simulink model "nb_spectrometer_17"  (R2012b)
(part 2 of 148)

      mask prompts: PFBSize "Size of PFB: (2^? pnts)"; TotalTaps "Total Number of Taps:"; WindowType "Windowing Function:"; n_inputs "Number of Simultaneous Inputs: (2^?)"; MakeBiplex "Make Biplex?"; BitWidthIn "Input Bitwidth:"; BitWidthOut "Output Bitwidth:"; CoeffBitWidth "Coefficient Bitwidth:"; CoeffDistMem "Use Distributed Memory for Coeffs"; add_latency "Add Latency"; mult_latency "Mult Latency"; bram_latency "BRAM Latency"; fan_latency "Fanout latency"; conv_latency "Convert latency"; quantization "Quantization Behavior"; fwidth "Bin Width Scaling (normal=1)"; mult_spec "Multiplier specification (0=core, 1=embedded, 2=behavioural) (left=1st tap, or just one value)"; adder_folding "Fold adders into DSPs"; adder_imp "Adder implementation"; coeffs_share "Share coefficients between polarisations (use less BRAM)?"
      mask help:
      | Fold adders into DSPs: Causes adders to be absorbed into DSP blocks (supported in Virtex5)
      | Adder implementation: Cores using Fabric or DSP48 or behavioral HDL
      mask init:
      | pfb_fir_real_init(gcb, ...
      |     'PFBSize', PFBSize, ...
      |     'TotalTaps', TotalTaps, ...
      |     'WindowType', WindowType, ...
      |     'n_inputs', n_inputs, ...
      |     'MakeBiplex', MakeBiplex, ...
      |     'BitWidthIn', BitWidthIn, ...
      |     'BitWidthOut', BitWidthOut, ...
      |     'CoeffBitWidth', CoeffBitWidth, ...
      |     'CoeffDistMem', CoeffDistMem, ...
      |     'add_latency', add_latency, ...
      |     'mult_latency', mult_latency, ...
      |     'bram_latency', bram_latency, ...
      |     'fan_latency', fan_latency, ...
      |     'conv_latency', conv_latency, ...
      |     'quantization', quantization, ...
      |     'fwidth', fwidth, ...
      |     'mult_spec', mult_spec, ...
      |     'adder_folding', adder_folding, ...
      |     'adder_imp', adder_imp, ...
      |     'coeffs_share', coeffs_share);
      settings: AttributesFormatString=taps=2, add_latency=1
      mask Help: eval('xlWeb(''http://casper.berkeley.edu/wiki/Pfb_fir_real'')')
      mask Callback TotalTaps:
      | %num_taps = eval(get_param(gcb, 'TotalTaps'));
      | %old_vec = eval(get_param(gcb, 'mult_spec'));=-0l
      | 
      | %vec = 2.*ones(1,num_taps);
      | %old_size = length(old_vec);
      | 
      | %if(old_size <= num_taps),
      | %    new_size = old_size;
      | %else,
      | %    new_size = num_taps;
      | %end
      | 
      | %for n = 1:new_size, vec(n) = old_vec(n); end
      | %set_param(gcb, 'mult_spec', mat2str(vec));
      mask TypeOptions WindowType: bartlett | barthannwin | blackman | blackmanharris | bohamwin | chebwin | flattopwin | gausswin | hamming | hann | kaiser | nuttallwin | parzenwin | rectwin | tukeywin | triang | userwindow
      mask TypeOptions quantization: Truncate | Round  (unbiased: +/- Inf) | Round  (unbiased: Even Values)
      mask TypeOptions adder_imp: Behavioral | Fabric | DSP48
  pfb_fir_real1 : Subsystem  Tag=casper:pfb_fir_real  AncestorBlock=casper_library_pfbs/pfb_fir_real  mask(pfb_fir_real){PFBSize=9, TotalTaps=2, WindowType=hamming, n_inputs=2, MakeBiplex=off, BitWidthIn=8, BitWidthOut=18, CoeffBitWidth=18, CoeffDistMem=off, add_latency=1, mult_latency=2, bram_latency=2, fan_latency=1, conv_latency=1, quantization=Round  (unbiased: Even Values), fwidth=1, mult_spec=2, adder_folding=on, adder_imp=Fabric, coeffs_share=off}
      mask prompts: PFBSize "Size of PFB: (2^? pnts)"; TotalTaps "Total Number of Taps:"; WindowType "Windowing Function:"; n_inputs "Number of Simultaneous Inputs: (2^?)"; MakeBiplex "Make Biplex?"; BitWidthIn "Input Bitwidth:"; BitWidthOut "Output Bitwidth:"; CoeffBitWidth "Coefficient Bitwidth:"; CoeffDistMem "Use Distributed Memory for Coeffs"; add_latency "Add Latency"; mult_latency "Mult Latency"; bram_latency "BRAM Latency"; fan_latency "Fanout latency"; conv_latency "Convert latency"; quantization "Quantization Behavior"; fwidth "Bin Width Scaling (normal=1)"; mult_spec "Multiplier specification (0=core, 1=embedded, 2=behavioural) (left=1st tap, or just one value)"; adder_folding "Fold adders into DSPs"; adder_imp "Adder implementation"; coeffs_share "Share coefficients between polarisations (use less BRAM)?"
      mask help:
      | Fold adders into DSPs: Causes adders to be absorbed into DSP blocks (supported in Virtex5)
      | Adder implementation: Cores using Fabric or DSP48 or behavioral HDL
      mask init: same as nb_spectrometer_17/pfb_fir_real
      settings: AttributesFormatString=taps=2, add_latency=1
      mask Help: eval('xlWeb(''http://casper.berkeley.edu/wiki/Pfb_fir_real'')')
      mask Callback TotalTaps:
      | %num_taps = eval(get_param(gcb, 'TotalTaps'));
      | %old_vec = eval(get_param(gcb, 'mult_spec'));=-0l
      | 
      | %vec = 2.*ones(1,num_taps);
      | %old_size = length(old_vec);
      | 
      | %if(old_size <= num_taps),
      | %    new_size = old_size;
      | %else,
      | %    new_size = num_taps;
      | %end
      | 
      | %for n = 1:new_size, vec(n) = old_vec(n); end
      | %set_param(gcb, 'mult_spec', mat2str(vec));
      mask TypeOptions WindowType: bartlett | barthannwin | blackman | blackmanharris | bohamwin | chebwin | flattopwin | gausswin | hamming | hann | kaiser | nuttallwin | parzenwin | rectwin | tukeywin | triang | userwindow
      mask TypeOptions quantization: Truncate | Round  (unbiased: +/- Inf) | Round  (unbiased: Even Values)
      mask TypeOptions adder_imp: Behavioral | Fabric | DSP48
  posedge : Subsystem  AncestorBlock=casper_library_misc/edge_detect  mask(edge_detect){edge=Rising, polarity=Active High, x_in=[0 0.08 0.08 0.16 0.16 0.24 0.24 0.32 0.32 0.4], y_in=[-1 -1  1  1  1  1  1  1  1  1], x_out=[0.6 0.68 0.68 0.76 0.76 0.84 0.84 0.92 0.92 1], y_out=[-1 -1  1  1 -1 -1 -1 -1 -1 -1]}
      mask prompts: edge "Edge Type"; polarity "Output Polarity"; x_in "Input X Positions"; y_in "Input Y Positions"; x_out "Output X Positions"; y_out "Output Y Positions"
      mask help: Output is active for one-cycle after each edge of the specified type (i.e. rising, falling or both).
      mask init:
      | edge_detect_init(gcb,...
      |     'edge',edge,...
      |     'polarity',polarity,...
      |     'x_in',x_in,...
      |     'x_out',x_out,...
      |     'y_in',y_in,...
      |     'y_out',y_out);
      | 
      | x_in_num=str2num(getfield(getfield(get_param(gcb,'UserData'),'parameters'),'x_in'));
      | x_out_num=str2num(getfield(getfield(get_param(gcb,'UserData'),'parameters'),'x_out'));
      | y_in_num=str2num(getfield(getfield(get_param(gcb,'UserData'),'parameters'),'y_in'));
      | y_out_num=str2num(getfield(getfield(get_param(gcb,'UserData'),'parameters'),'y_out'));
      settings: AttributesFormatString=|
      | rising edges
      | active high
      mask Help: Output is active for one-cycle after each edge of the specified type (i.e. rising, falling, or both).  Latency is zero.
      mask TypeOptions edge: Rising | Falling | Both
      mask TypeOptions polarity: Active High | Active Low
      mask Display:
      | plot(x_in_num,0.5+y_in_num*0.2);
      | plot(x_out_num,0.5+y_out_num*0.2);
  posedge1 : Subsystem  AncestorBlock=casper_library_misc/edge_detect  mask(edge_detect){edge=Rising, polarity=Active High, x_in=[0 0.08 0.08 0.16 0.16 0.24 0.24 0.32 0.32 0.4], y_in=[-1 -1  1  1  1  1  1  1  1  1], x_out=[0.6 0.68 0.68 0.76 0.76 0.84 0.84 0.92 0.92 1], y_out=[-1 -1  1  1 -1 -1 -1 -1 -1 -1]}
      mask prompts: edge "Edge Type"; polarity "Output Polarity"; x_in "Input X Positions"; y_in "Input Y Positions"; x_out "Output X Positions"; y_out "Output Y Positions"
      mask help: Output is active for one-cycle after each edge of the specified type (i.e. rising, falling or both).
      mask init: same as nb_spectrometer_17/posedge
      settings: AttributesFormatString=|
      | rising edges
      | active high
      mask Help: Output is active for one-cycle after each edge of the specified type (i.e. rising, falling, or both).  Latency is zero.
      mask TypeOptions edge: Rising | Falling | Both
      mask TypeOptions polarity: Active High | Active Low
      mask Display:
      | plot(x_in_num,0.5+y_in_num*0.2);
      | plot(x_out_num,0.5+y_out_num*0.2);
  posedge10 : Subsystem  AncestorBlock=casper_library_misc/edge_detect  mask(edge_detect){edge=Rising, polarity=Active High, x_in=[0 0.08 0.08 0.16 0.16 0.24 0.24 0.32 0.32 0.4], y_in=[-1 -1  1  1  1  1  1  1  1  1], x_out=[0.6 0.68 0.68 0.76 0.76 0.84 0.84 0.92 0.92 1], y_out=[-1 -1  1  1 -1 -1 -1 -1 -1 -1]}
      mask prompts: edge "Edge Type"; polarity "Output Polarity"; x_in "Input X Positions"; y_in "Input Y Positions"; x_out "Output X Positions"; y_out "Output Y Positions"
      mask help: Output is active for one-cycle after each edge of the specified type (i.e. rising, falling or both).
      mask init: same as nb_spectrometer_17/posedge
      settings: AttributesFormatString=|
      | rising edges
      | active high
      mask Help: Output is active for one-cycle after each edge of the specified type (i.e. rising, falling, or both).  Latency is zero.
      mask TypeOptions edge: Rising | Falling | Both
      mask TypeOptions polarity: Active High | Active Low
      mask Display:
      | plot(x_in_num,0.5+y_in_num*0.2);
      | plot(x_out_num,0.5+y_out_num*0.2);
  posedge11 : Subsystem  AncestorBlock=casper_library_misc/edge_detect  mask(edge_detect){edge=Rising, polarity=Active High, x_in=[0 0.08 0.08 0.16 0.16 0.24 0.24 0.32 0.32 0.4], y_in=[-1 -1  1  1  1  1  1  1  1  1], x_out=[0.6 0.68 0.68 0.76 0.76 0.84 0.84 0.92 0.92 1], y_out=[-1 -1  1  1 -1 -1 -1 -1 -1 -1]}
      mask prompts: edge "Edge Type"; polarity "Output Polarity"; x_in "Input X Positions"; y_in "Input Y Positions"; x_out "Output X Positions"; y_out "Output Y Positions"
      mask help: Output is active for one-cycle after each edge of the specified type (i.e. rising, falling or both).
      mask init: same as nb_spectrometer_17/posedge
      settings: AttributesFormatString=|
      | rising edges
      | active high
      mask Help: Output is active for one-cycle after each edge of the specified type (i.e. rising, falling, or both).  Latency is zero.
      mask TypeOptions edge: Rising | Falling | Both
      mask TypeOptions polarity: Active High | Active Low
      mask Display:
      | plot(x_in_num,0.5+y_in_num*0.2);
      | plot(x_out_num,0.5+y_out_num*0.2);
  posedge12 : Subsystem  AncestorBlock=casper_library_misc/edge_detect  mask(edge_detect){edge=Rising, polarity=Active High, x_in=[0 0.08 0.08 0.16 0.16 0.24 0.24 0.32 0.32 0.4], y_in=[-1 -1  1  1  1  1  1  1  1  1], x_out=[0.6 0.68 0.68 0.76 0.76 0.84 0.84 0.92 0.92 1], y_out=[-1 -1  1  1 -1 -1 -1 -1 -1 -1]}
      mask prompts: edge "Edge Type"; polarity "Output Polarity"; x_in "Input X Positions"; y_in "Input Y Positions"; x_out "Output X Positions"; y_out "Output Y Positions"
      mask help: Output is active for one-cycle after each edge of the specified type (i.e. rising, falling or both).
      mask init: same as nb_spectrometer_17/posedge
      settings: AttributesFormatString=|
      | rising edges
      | active high
      mask Help: Output is active for one-cycle after each edge of the specified type (i.e. rising, falling, or both).  Latency is zero.
      mask TypeOptions edge: Rising | Falling | Both
      mask TypeOptions polarity: Active High | Active Low
      mask Display:
      | plot(x_in_num,0.5+y_in_num*0.2);
      | plot(x_out_num,0.5+y_out_num*0.2);
  posedge13 : Subsystem  AncestorBlock=casper_library_misc/edge_detect  mask(edge_detect){edge=Rising, polarity=Active High, x_in=[0 0.08 0.08 0.16 0.16 0.24 0.24 0.32 0.32 0.4], y_in=[-1 -1  1  1  1  1  1  1  1  1], x_out=[0.6 0.68 0.68 0.76 0.76 0.84 0.84 0.92 0.92 1], y_out=[-1 -1  1  1 -1 -1 -1 -1 -1 -1]}
      mask prompts: edge "Edge Type"; polarity "Output Polarity"; x_in "Input X Positions"; y_in "Input Y Positions"; x_out "Output X Positions"; y_out "Output Y Positions"
      mask help: Output is active for one-cycle after each edge of the specified type (i.e. rising, falling or both).
      mask init: same as nb_spectrometer_17/posedge
      settings: AttributesFormatString=|
      | rising edges
      | active high
      mask Help: Output is active for one-cycle after each edge of the specified type (i.e. rising, falling, or both).  Latency is zero.
      mask TypeOptions edge: Rising | Falling | Both
      mask TypeOptions polarity: Active High | Active Low
      mask Display:
      | plot(x_in_num,0.5+y_in_num*0.2);
      | plot(x_out_num,0.5+y_out_num*0.2);
  posedge14 : Subsystem  AncestorBlock=casper_library_misc/edge_detect  mask(edge_detect){edge=Rising, polarity=Active High, x_in=[0 0.08 0.08 0.16 0.16 0.24 0.24 0.32 0.32 0.4], y_in=[-1 -1  1  1  1  1  1  1  1  1], x_out=[0.6 0.68 0.68 0.76 0.76 0.84 0.84 0.92 0.92 1], y_out=[-1 -1  1  1 -1 -1 -1 -1 -1 -1]}
      mask prompts: edge "Edge Type"; polarity "Output Polarity"; x_in "Input X Positions"; y_in "Input Y Positions"; x_out "Output X Positions"; y_out "Output Y Positions"
      mask help: Output is active for one-cycle after each edge of the specified type (i.e. rising, falling or both).
      mask init: same as nb_spectrometer_17/posedge
      settings: AttributesFormatString=|
      | rising edges
      | active high
      mask Help: Output is active for one-cycle after each edge of the specified type (i.e. rising, falling, or both).  Latency is zero.
      mask TypeOptions edge: Rising | Falling | Both
      mask TypeOptions polarity: Active High | Active Low
      mask Display:
      | plot(x_in_num,0.5+y_in_num*0.2);
      | plot(x_out_num,0.5+y_out_num*0.2);
  posedge15 : Subsystem  AncestorBlock=casper_library_misc/edge_detect  mask(edge_detect){edge=Rising, polarity=Active High, x_in=[0 0.08 0.08 0.16 0.16 0.24 0.24 0.32 0.32 0.4], y_in=[-1 -1  1  1  1  1  1  1  1  1], x_out=[0.6 0.68 0.68 0.76 0.76 0.84 0.84 0.92 0.92 1], y_out=[-1 -1  1  1 -1 -1 -1 -1 -1 -1]}
      mask prompts: edge "Edge Type"; polarity "Output Polarity"; x_in "Input X Positions"; y_in "Input Y Positions"; x_out "Output X Positions"; y_out "Output Y Positions"
      mask help: Output is active for one-cycle after each edge of the specified type (i.e. rising, falling or both).
      mask init: same as nb_spectrometer_17/posedge
      settings: AttributesFormatString=|
      | rising edges
      | active high
      mask Help: Output is active for one-cycle after each edge of the specified type (i.e. rising, falling, or both).  Latency is zero.
      mask TypeOptions edge: Rising | Falling | Both
      mask TypeOptions polarity: Active High | Active Low
      mask Display:
      | plot(x_in_num,0.5+y_in_num*0.2);
      | plot(x_out_num,0.5+y_out_num*0.2);
  posedge16 : Subsystem  AncestorBlock=casper_library_misc/edge_detect  mask(edge_detect){edge=Rising, polarity=Active High, x_in=[0 0.08 0.08 0.16 0.16 0.24 0.24 0.32 0.32 0.4], y_in=[-1 -1  1  1  1  1  1  1  1  1], x_out=[0.6 0.68 0.68 0.76 0.76 0.84 0.84 0.92 0.92 1], y_out=[-1 -1  1  1 -1 -1 -1 -1 -1 -1]}
      mask prompts: edge "Edge Type"; polarity "Output Polarity"; x_in "Input X Positions"; y_in "Input Y Positions"; x_out "Output X Positions"; y_out "Output Y Positions"
      mask help: Output is active for one-cycle after each edge of the specified type (i.e. rising, falling or both).
      mask init: same as nb_spectrometer_17/posedge
      settings: AttributesFormatString=|
      | rising edges
      | active high
      mask Help: Output is active for one-cycle after each edge of the specified type (i.e. rising, falling, or both).  Latency is zero.
      mask TypeOptions edge: Rising | Falling | Both
      mask TypeOptions polarity: Active High | Active Low
      mask Display:
      | plot(x_in_num,0.5+y_in_num*0.2);
      | plot(x_out_num,0.5+y_out_num*0.2);
  posedge17 : Subsystem  AncestorBlock=casper_library_misc/edge_detect  mask(edge_detect){edge=Falling, polarity=Active High, x_in=[0 0.08 0.08 0.16 0.16 0.24 0.24 0.32 0.32 0.4], y_in=[-1 -1  1  1  1  1  1  1  1  1], x_out=[0.6 0.68 0.68 0.76 0.76 0.84 0.84 0.92 0.92 1], y_out=[-1 -1  1  1 -1 -1 -1 -1 -1 -1]}
      mask prompts: edge "Edge Type"; polarity "Output Polarity"; x_in "Input X Positions"; y_in "Input Y Positions"; x_out "Output X Positions"; y_out "Output Y Positions"
      mask help: Output is active for one-cycle after each edge of the specified type (i.e. rising, falling or both).
      mask init: same as nb_spectrometer_17/posedge
      settings: AttributesFormatString=|
      | falling edges
      | active high
      mask Help: Output is active for one-cycle after each edge of the specified type (i.e. rising, falling, or both).  Latency is zero.
      mask TypeOptions edge: Rising | Falling | Both
      mask TypeOptions polarity: Active High | Active Low
      mask Display:
      | plot(x_in_num,0.5+y_in_num*0.2);
      | plot(x_out_num,0.5+y_out_num*0.2);
  posedge18 : Subsystem  AncestorBlock=casper_library_misc/edge_detect  mask(edge_detect){edge=Rising, polarity=Active High, x_in=[0 0.08 0.08 0.16 0.16 0.24 0.24 0.32 0.32 0.4], y_in=[-1 -1  1  1  1  1  1  1  1  1], x_out=[0.6 0.68 0.68 0.76 0.76 0.84 0.84 0.92 0.92 1], y_out=[-1 -1  1  1 -1 -1 -1 -1 -1 -1]}
      mask prompts: edge "Edge Type"; polarity "Output Polarity"; x_in "Input X Positions"; y_in "Input Y Positions"; x_out "Output X Positions"; y_out "Output Y Positions"
      mask help: Output is active for one-cycle after each edge of the specified type (i.e. rising, falling or both).
      mask init: same as nb_spectrometer_17/posedge
      settings: AttributesFormatString=|
      | rising edges
      | active high
      mask Help: Output is active for one-cycle after each edge of the specified type (i.e. rising, falling, or both).  Latency is zero.
      mask TypeOptions edge: Rising | Falling | Both
      mask TypeOptions polarity: Active High | Active Low
      mask Display:
      | plot(x_in_num,0.5+y_in_num*0.2);
      | plot(x_out_num,0.5+y_out_num*0.2);
  posedge19 : Subsystem  AncestorBlock=casper_library_misc/edge_detect  mask(edge_detect){edge=Rising, polarity=Active High, x_in=[0 0.08 0.08 0.16 0.16 0.24 0.24 0.32 0.32 0.4], y_in=[-1 -1  1  1  1  1  1  1  1  1], x_out=[0.6 0.68 0.68 0.76 0.76 0.84 0.84 0.92 0.92 1], y_out=[-1 -1  1  1 -1 -1 -1 -1 -1 -1]}
      mask prompts: edge "Edge Type"; polarity "Output Polarity"; x_in "Input X Positions"; y_in "Input Y Positions"; x_out "Output X Positions"; y_out "Output Y Positions"
      mask help: Output is active for one-cycle after each edge of the specified type (i.e. rising, falling or both).
      mask init: same as nb_spectrometer_17/posedge
      settings: AttributesFormatString=|
      | rising edges
      | active high
      mask Help: Output is active for one-cycle after each edge of the specified type (i.e. rising, falling, or both).  Latency is zero.
      mask TypeOptions edge: Rising | Falling | Both
      mask TypeOptions polarity: Active High | Active Low
      mask Display:
      | plot(x_in_num,0.5+y_in_num*0.2);
      | plot(x_out_num,0.5+y_out_num*0.2);
  posedge2 : Subsystem  AncestorBlock=casper_library_misc/edge_detect  mask(edge_detect){edge=Rising, polarity=Active High, x_in=[0 0.08 0.08 0.16 0.16 0.24 0.24 0.32 0.32 0.4], y_in=[-1 -1  1  1  1  1  1  1  1  1], x_out=[0.6 0.68 0.68 0.76 0.76 0.84 0.84 0.92 0.92 1], y_out=[-1 -1  1  1 -1 -1 -1 -1 -1 -1]}
      mask prompts: edge "Edge Type"; polarity "Output Polarity"; x_in "Input X Positions"; y_in "Input Y Positions"; x_out "Output X Positions"; y_out "Output Y Positions"
      mask help: Output is active for one-cycle after each edge of the specified type (i.e. rising, falling or both).
      mask init: same as nb_spectrometer_17/posedge
      settings: AttributesFormatString=|
      | rising edges
      | active high
      mask Help: Output is active for one-cycle after each edge of the specified type (i.e. rising, falling, or both).  Latency is zero.
      mask TypeOptions edge: Rising | Falling | Both
      mask TypeOptions polarity: Active High | Active Low
      mask Display:
      | plot(x_in_num,0.5+y_in_num*0.2);
      | plot(x_out_num,0.5+y_out_num*0.2);
  posedge20 : Subsystem  AncestorBlock=casper_library_misc/edge_detect  mask(edge_detect){edge=Rising, polarity=Active High, x_in=[0 0.08 0.08 0.16 0.16 0.24 0.24 0.32 0.32 0.4], y_in=[-1 -1  1  1  1  1  1  1  1  1], x_out=[0.6 0.68 0.68 0.76 0.76 0.84 0.84 0.92 0.92 1], y_out=[-1 -1  1  1 -1 -1 -1 -1 -1 -1]}
      mask prompts: edge "Edge Type"; polarity "Output Polarity"; x_in "Input X Positions"; y_in "Input Y Positions"; x_out "Output X Positions"; y_out "Output Y Positions"
      mask help: Output is active for one-cycle after each edge of the specified type (i.e. rising, falling or both).
      mask init: same as nb_spectrometer_17/posedge
      settings: AttributesFormatString=|
      | rising edges
      | active high
      mask Help: Output is active for one-cycle after each edge of the specified type (i.e. rising, falling, or both).  Latency is zero.
      mask TypeOptions edge: Rising | Falling | Both
      mask TypeOptions polarity: Active High | Active Low
      mask Display:
      | plot(x_in_num,0.5+y_in_num*0.2);
      | plot(x_out_num,0.5+y_out_num*0.2);
  posedge3 : Subsystem  AncestorBlock=casper_library_misc/edge_detect  mask(edge_detect){edge=Rising, polarity=Active High, x_in=[0 0.08 0.08 0.16 0.16 0.24 0.24 0.32 0.32 0.4], y_in=[-1 -1  1  1  1  1  1  1  1  1], x_out=[0.6 0.68 0.68 0.76 0.76 0.84 0.84 0.92 0.92 1], y_out=[-1 -1  1  1 -1 -1 -1 -1 -1 -1]}
      mask prompts: edge "Edge Type"; polarity "Output Polarity"; x_in "Input X Positions"; y_in "Input Y Positions"; x_out "Output X Positions"; y_out "Output Y Positions"
      mask help: Output is active for one-cycle after each edge of the specified type (i.e. rising, falling or both).
      mask init: same as nb_spectrometer_17/posedge
      settings: AttributesFormatString=|
      | rising edges
      | active high
      mask Help: Output is active for one-cycle after each edge of the specified type (i.e. rising, falling, or both).  Latency is zero.
      mask TypeOptions edge: Rising | Falling | Both
      mask TypeOptions polarity: Active High | Active Low
      mask Display:
      | plot(x_in_num,0.5+y_in_num*0.2);
      | plot(x_out_num,0.5+y_out_num*0.2);
  posedge4 : Subsystem  AncestorBlock=casper_library_misc/edge_detect  mask(edge_detect){edge=Rising, polarity=Active High, x_in=[0 0.08 0.08 0.16 0.16 0.24 0.24 0.32 0.32 0.4], y_in=[-1 -1  1  1  1  1  1  1  1  1], x_out=[0.6 0.68 0.68 0.76 0.76 0.84 0.84 0.92 0.92 1], y_out=[-1 -1  1  1 -1 -1 -1 -1 -1 -1]}
      mask prompts: edge "Edge Type"; polarity "Output Polarity"; x_in "Input X Positions"; y_in "Input Y Positions"; x_out "Output X Positions"; y_out "Output Y Positions"
      mask help: Output is active for one-cycle after each edge of the specified type (i.e. rising, falling or both).
      mask init: same as nb_spectrometer_17/posedge
      settings: AttributesFormatString=|
      | rising edges
      | active high
      mask Help: Output is active for one-cycle after each edge of the specified type (i.e. rising, falling, or both).  Latency is zero.
      mask TypeOptions edge: Rising | Falling | Both
      mask TypeOptions polarity: Active High | Active Low
      mask Display:
      | plot(x_in_num,0.5+y_in_num*0.2);
      | plot(x_out_num,0.5+y_out_num*0.2);
  posedge5 : Subsystem  AncestorBlock=casper_library_misc/edge_detect  mask(edge_detect){edge=Rising, polarity=Active High, x_in=[0 0.08 0.08 0.16 0.16 0.24 0.24 0.32 0.32 0.4], y_in=[-1 -1  1  1  1  1  1  1  1  1], x_out=[0.6 0.68 0.68 0.76 0.76 0.84 0.84 0.92 0.92 1], y_out=[-1 -1  1  1 -1 -1 -1 -1 -1 -1]}
      mask prompts: edge "Edge Type"; polarity "Output Polarity"; x_in "Input X Positions"; y_in "Input Y Positions"; x_out "Output X Positions"; y_out "Output Y Positions"
      mask help: Output is active for one-cycle after each edge of the specified type (i.e. rising, falling or both).
      mask init: same as nb_spectrometer_17/posedge
      settings: AttributesFormatString=|
      | rising edges
      | active high
      mask Help: Output is active for one-cycle after each edge of the specified type (i.e. rising, falling, or both).  Latency is zero.
      mask TypeOptions edge: Rising | Falling | Both
      mask TypeOptions polarity: Active High | Active Low
      mask Display:
      | plot(x_in_num,0.5+y_in_num*0.2);
      | plot(x_out_num,0.5+y_out_num*0.2);
  posedge6 : Subsystem  AncestorBlock=casper_library_misc/edge_detect  mask(edge_detect){edge=Rising, polarity=Active High, x_in=[0 0.08 0.08 0.16 0.16 0.24 0.24 0.32 0.32 0.4], y_in=[-1 -1  1  1  1  1  1  1  1  1], x_out=[0.6 0.68 0.68 0.76 0.76 0.84 0.84 0.92 0.92 1], y_out=[-1 -1  1  1 -1 -1 -1 -1 -1 -1]}
      mask prompts: edge "Edge Type"; polarity "Output Polarity"; x_in "Input X Positions"; y_in "Input Y Positions"; x_out "Output X Positions"; y_out "Output Y Positions"
      mask help: Output is active for one-cycle after each edge of the specified type (i.e. rising, falling or both).
      mask init: same as nb_spectrometer_17/posedge
      settings: AttributesFormatString=|
      | rising edges
      | active high
      mask Help: Output is active for one-cycle after each edge of the specified type (i.e. rising, falling, or both).  Latency is zero.
      mask TypeOptions edge: Rising | Falling | Both
      mask TypeOptions polarity: Active High | Active Low
      mask Display:
      | plot(x_in_num,0.5+y_in_num*0.2);
      | plot(x_out_num,0.5+y_out_num*0.2);
  posedge7 : Subsystem  AncestorBlock=casper_library_misc/edge_detect  mask(edge_detect){edge=Rising, polarity=Active High, x_in=[0 0.08 0.08 0.16 0.16 0.24 0.24 0.32 0.32 0.4], y_in=[-1 -1  1  1  1  1  1  1  1  1], x_out=[0.6 0.68 0.68 0.76 0.76 0.84 0.84 0.92 0.92 1], y_out=[-1 -1  1  1 -1 -1 -1 -1 -1 -1]}
      mask prompts: edge "Edge Type"; polarity "Output Polarity"; x_in "Input X Positions"; y_in "Input Y Positions"; x_out "Output X Positions"; y_out "Output Y Positions"
      mask help: Output is active for one-cycle after each edge of the specified type (i.e. rising, falling or both).
      mask init: same as nb_spectrometer_17/posedge
      settings: AttributesFormatString=|
      | rising edges
      | active high
      mask Help: Output is active for one-cycle after each edge of the specified type (i.e. rising, falling, or both).  Latency is zero.
      mask TypeOptions edge: Rising | Falling | Both
      mask TypeOptions polarity: Active High | Active Low
      mask Display:
      | plot(x_in_num,0.5+y_in_num*0.2);
      | plot(x_out_num,0.5+y_out_num*0.2);
  posedge8 : Subsystem  AncestorBlock=casper_library_misc/edge_detect  mask(edge_detect){edge=Rising, polarity=Active High, x_in=[0 0.08 0.08 0.16 0.16 0.24 0.24 0.32 0.32 0.4], y_in=[-1 -1  1  1  1  1  1  1  1  1], x_out=[0.6 0.68 0.68 0.76 0.76 0.84 0.84 0.92 0.92 1], y_out=[-1 -1  1  1 -1 -1 -1 -1 -1 -1]}
      mask prompts: edge "Edge Type"; polarity "Output Polarity"; x_in "Input X Positions"; y_in "Input Y Positions"; x_out "Output X Positions"; y_out "Output Y Positions"
      mask help: Output is active for one-cycle after each edge of the specified type (i.e. rising, falling or both).
      mask init: same as nb_spectrometer_17/posedge
      settings: AttributesFormatString=|
      | rising edges
      | active high
      mask Help: Output is active for one-cycle after each edge of the specified type (i.e. rising, falling, or both).  Latency is zero.
      mask TypeOptions edge: Rising | Falling | Both
      mask TypeOptions polarity: Active High | Active Low
      mask Display:
      | plot(x_in_num,0.5+y_in_num*0.2);
      | plot(x_out_num,0.5+y_out_num*0.2);
  posedge9 : Subsystem  AncestorBlock=casper_library_misc/edge_detect  mask(edge_detect){edge=Rising, polarity=Active High, x_in=[0 0.08 0.08 0.16 0.16 0.24 0.24 0.32 0.32 0.4], y_in=[-1 -1  1  1  1  1  1  1  1  1], x_out=[0.6 0.68 0.68 0.76 0.76 0.84 0.84 0.92 0.92 1], y_out=[-1 -1  1  1 -1 -1 -1 -1 -1 -1]}
      mask prompts: edge "Edge Type"; polarity "Output Polarity"; x_in "Input X Positions"; y_in "Input Y Positions"; x_out "Output X Positions"; y_out "Output Y Positions"
      mask help: Output is active for one-cycle after each edge of the specified type (i.e. rising, falling or both).
      mask init: same as nb_spectrometer_17/posedge
      settings: AttributesFormatString=|
      | rising edges
      | active high
      mask Help: Output is active for one-cycle after each edge of the specified type (i.e. rising, falling, or both).  Latency is zero.
      mask TypeOptions edge: Rising | Falling | Both
      mask TypeOptions polarity: Active High | Active Low
      mask Display:
      | plot(x_in_num,0.5+y_in_num*0.2);
      | plot(x_out_num,0.5+y_out_num*0.2);
  pps_cnt : Subsystem  Tag=xps:sw_reg  AncestorBlock=xps_library/software register  mask(swreg){mode=one value, io_dir=To Processor, io_delay=0, sample_period=1, names=reg, bitwidths=32, arith_types=0, bin_pts=0, sim_port=on, show_format=off}
      mask prompts: io_dir "I/O direction"; io_delay "I/O delay"; sample_period "Sample period"; names "Name:"; bitwidths "Bitwidth:"; arith_types "Type (ufix=0, fix=1, bool=2):"; bin_pts "Binary pt:"; sim_port "Provide sim input/output?"; show_format "Print format string?"
      mask init:
      | swreg_init(gcb)
      settings: AttributesFormatString=1output
      mask TypeOptions mode: one value | fields of equal size | fields of arbitrary size
      mask Callback mode: swreg_cb(gcb);
      mask TypeOptions io_dir: To Processor | From Processor
      mask Callback io_dir:
      | mask_enables = get_param(gcb, 'MaskEnables');
      | mask_names = get_param(gcb, 'MaskNames');
      | if strcmp(get_param(gcb, 'io_dir'), 'To Processor'),
      |     mask_enables{ismember(mask_names, 'sample_period')} = 'off';
      | else
      |     mask_enables{ismember(mask_names, 'sample_period')} = 'on';
      | end
      | set_param(gcb, 'MaskEnables', mask_enables);
      mask Callback bitwidths: swreg_maskcheck(gcb);
      mask Callback arith_types: [numios, ~, ~, ~, current_types] = swreg_maskcheck(gcb);
      mask Callback bin_pts: swreg_maskcheck(gcb);
  pps_cnt1 : Subsystem  Tag=xps:sw_reg  Commented=on  AncestorBlock=xps_library/software register  mask(swreg){mode=one value, io_dir=To Processor, io_delay=0, sample_period=1, names=reg, bitwidths=32, arith_types=0, bin_pts=0, sim_port=on, show_format=off}
      mask prompts: io_dir "I/O direction"; io_delay "I/O delay"; sample_period "Sample period"; names "Name:"; bitwidths "Bitwidth:"; arith_types "Type (ufix=0, fix=1, bool=2):"; bin_pts "Binary pt:"; sim_port "Provide sim input/output?"; show_format "Print format string?"
      mask init:
      | swreg_init(gcb)
      settings: AttributesFormatString=1output
      mask TypeOptions mode: one value | fields of equal size | fields of arbitrary size
      mask Callback mode: swreg_cb(gcb);
      mask TypeOptions io_dir: To Processor | From Processor
      mask Callback io_dir:
      | mask_enables = get_param(gcb, 'MaskEnables');
      | mask_names = get_param(gcb, 'MaskNames');
      | if strcmp(get_param(gcb, 'io_dir'), 'To Processor'),
      |     mask_enables{ismember(mask_names, 'sample_period')} = 'off';
      | else
      |     mask_enables{ismember(mask_names, 'sample_period')} = 'on';
      | end
      | set_param(gcb, 'MaskEnables', mask_enables);
      mask Callback bitwidths: swreg_maskcheck(gcb);
      mask Callback arith_types: [numios, ~, ~, ~, current_types] = swreg_maskcheck(gcb);
      mask Callback bin_pts: swreg_maskcheck(gcb);
  pulse_ext{,1..6} (7 alike) : casper_library_misc/pulse_ext  pulse_len=20000000
  queue_empty : Subsystem  Tag=xps:sw_reg  AncestorBlock=xps_library/software register  mask(swreg){mode=one value, io_dir=To Processor, io_delay=0, sample_period=1, names=reg, bitwidths=1, arith_types=2, bin_pts=0, sim_port=on, show_format=off}
      mask prompts: io_dir "I/O direction"; io_delay "I/O delay"; sample_period "Sample period"; names "Name:"; bitwidths "Bitwidth:"; arith_types "Type (ufix=0, fix=1, bool=2):"; bin_pts "Binary pt:"; sim_port "Provide sim input/output?"; show_format "Print format string?"
      mask init:
      | swreg_init(gcb)
      settings: AttributesFormatString=1output
      mask TypeOptions mode: one value | fields of equal size | fields of arbitrary size
      mask Callback mode: swreg_cb(gcb);
      mask TypeOptions io_dir: To Processor | From Processor
      mask Callback io_dir:
      | mask_enables = get_param(gcb, 'MaskEnables');
      | mask_names = get_param(gcb, 'MaskNames');
      | if strcmp(get_param(gcb, 'io_dir'), 'To Processor'),
      |     mask_enables{ismember(mask_names, 'sample_period')} = 'off';
      | else
      |     mask_enables{ismember(mask_names, 'sample_period')} = 'on';
      | end
      | set_param(gcb, 'MaskEnables', mask_enables);
      mask Callback bitwidths: swreg_maskcheck(gcb);
      mask Callback arith_types: [numios, ~, ~, ~, current_types] = swreg_maskcheck(gcb);
      mask Callback bin_pts: swreg_maskcheck(gcb);
  queue_perc_full : Subsystem  Tag=xps:sw_reg  AncestorBlock=xps_library/software register  mask(swreg){mode=one value, io_dir=To Processor, io_delay=0, sample_period=1, names=reg, bitwidths=8, arith_types=0, bin_pts=8, sim_port=on, show_format=off}
      mask prompts: io_dir "I/O direction"; io_delay "I/O delay"; sample_period "Sample period"; names "Name:"; bitwidths "Bitwidth:"; arith_types "Type (ufix=0, fix=1, bool=2):"; bin_pts "Binary pt:"; sim_port "Provide sim input/output?"; show_format "Print format string?"
      mask init:
      | swreg_init(gcb)
      settings: AttributesFormatString=1output
      mask TypeOptions mode: one value | fields of equal size | fields of arbitrary size
      mask Callback mode: swreg_cb(gcb);
      mask TypeOptions io_dir: To Processor | From Processor
      mask Callback io_dir:
      | mask_enables = get_param(gcb, 'MaskEnables');
      | mask_names = get_param(gcb, 'MaskNames');
      | if strcmp(get_param(gcb, 'io_dir'), 'To Processor'),
      |     mask_enables{ismember(mask_names, 'sample_period')} = 'off';
      | else
      |     mask_enables{ismember(mask_names, 'sample_period')} = 'on';
      | end
      | set_param(gcb, 'MaskEnables', mask_enables);
      mask Callback bitwidths: swreg_maskcheck(gcb);
      mask Callback arith_types: [numios, ~, ~, ~, current_types] = swreg_maskcheck(gcb);
      mask Callback bin_pts: swreg_maskcheck(gcb);
  reinterpret10 : xbsIndex_r4/Reinterpret  force_arith_type=on  arith_type="Signed  (2's comp)"  force_bin_pt=on  bin_pt=0  block_type=reinterpret
  reinterpret11 : xbsIndex_r4/Reinterpret  force_arith_type=on  arith_type="Signed  (2's comp)"  force_bin_pt=on  bin_pt=0  block_type=reinterpret
  relational12 : xbsIndex_r4/Relational  mode=a>b  en=off  latency=1  dbl_ovrd=off  block_type=relational
  relational13 : xbsIndex_r4/Relational  mode=a<b  en=off  latency=1  dbl_ovrd=off  block_type=relational
  relational14 : xbsIndex_r4/Relational  mode=a>b  en=off  latency=0  dbl_ovrd=off  block_type=relational
  relational15 : xbsIndex_r4/Relational  mode=a>b  en=off  latency=1  dbl_ovrd=off  block_type=relational
  relational16 : xbsIndex_r4/Relational  mode=a<b  en=off  latency=1  dbl_ovrd=off  block_type=relational
  roach_gpio_a_enable_not : xps_library/gpio  Tag=xps:gpio  io_group=ROACH:gpioa_oe_n  io_dir=out  arith_type=Boolean  bitwidth=1  bin_pt=0  bit_index=0  sample_period=1  use_single_ended=off  use_ddr=off  reg_iob=off  reg_clk_phase=0  termination=None
      link override convert: arith_type=Boolean  n_bits=1  bin_pt=0
  roach_gpio_b_enable_not : xps_library/gpio  Tag=xps:gpio  io_group=ROACH:gpiob_oe_n  io_dir=out  arith_type=Boolean  bitwidth=1  bin_pt=0  bit_index=0  sample_period=1  use_single_ended=off  use_ddr=off  reg_iob=off  reg_clk_phase=0  termination=None
      link override convert: arith_type=Boolean  n_bits=1  bin_pt=0
  roach_led0 : xps_library/gpio  Tag=xps:gpio  io_group=ROACH:gpiob  io_dir=out  arith_type=Boolean  bitwidth=1  bin_pt=0  bit_index=0  sample_period=1  use_single_ended=off  use_ddr=off  reg_iob=off  reg_clk_phase=0  termination=None
      link override convert: arith_type=Boolean  n_bits=1  bin_pt=0
  roach_led1 : xps_library/gpio  Tag=xps:gpio  io_group=ROACH:gpiob  io_dir=out  arith_type=Boolean  bitwidth=1  bin_pt=0  bit_index=1  sample_period=1  use_single_ended=off  use_ddr=off  reg_iob=off  reg_clk_phase=0  termination=None
      link override convert: arith_type=Boolean  n_bits=1  bin_pt=0
  roach_led2 : xps_library/gpio  Tag=xps:gpio  io_group=ROACH:gpiob  io_dir=out  arith_type=Boolean  bitwidth=1  bin_pt=0  bit_index=2  sample_period=1  use_single_ended=off  use_ddr=off  reg_iob=off  reg_clk_phase=0  termination=None
      link override convert: arith_type=Boolean  n_bits=1  bin_pt=0
  roach_led3 : xps_library/gpio  Tag=xps:gpio  io_group=ROACH:gpiob  io_dir=out  arith_type=Boolean  bitwidth=1  bin_pt=0  bit_index=3  sample_period=1  use_single_ended=off  use_ddr=off  reg_iob=off  reg_clk_phase=0  termination=None
      link override convert: arith_type=Boolean  n_bits=1  bin_pt=0
  roach_led4 : xps_library/gpio  Tag=xps:gpio  io_group=ROACH:gpiob  io_dir=out  arith_type=Boolean  bitwidth=1  bin_pt=0  bit_index=4  sample_period=1  use_single_ended=off  use_ddr=off  reg_iob=off  reg_clk_phase=0  termination=None
      link override convert: arith_type=Boolean  n_bits=1  bin_pt=0
  roach_led5 : xps_library/gpio  Tag=xps:gpio  io_group=ROACH:gpiob  io_dir=out  arith_type=Boolean  bitwidth=1  bin_pt=0  bit_index=5  sample_period=1  use_single_ended=off  use_ddr=off  reg_iob=off  reg_clk_phase=0  termination=None
      link override convert: arith_type=Boolean  n_bits=1  bin_pt=0
  roach_led6 : xps_library/gpio  Tag=xps:gpio  io_group=ROACH:gpiob  io_dir=out  arith_type=Boolean  bitwidth=1  bin_pt=0  bit_index=6  sample_period=1  use_single_ended=off  use_ddr=off  reg_iob=off  reg_clk_phase=0  termination=None
      link override convert: arith_type=Boolean  n_bits=1  bin_pt=0
  roach_led7 : xps_library/gpio  Tag=xps:gpio  io_group=ROACH:gpiob  io_dir=out  arith_type=Boolean  bitwidth=1  bin_pt=0  bit_index=7  sample_period=1  use_single_ended=off  use_ddr=off  reg_iob=off  reg_clk_phase=0  termination=None
      link override convert: arith_type=Boolean  n_bits=1  bin_pt=0
  roach_sma_j10 : xps_library/gpio  Tag=xps:gpio  io_group=ROACH:gpioa  io_dir=out  arith_type=Boolean  bitwidth=1  bin_pt=0  bit_index=4  sample_period=1  use_single_ended=off  use_ddr=off  reg_iob=off  reg_clk_phase=0  termination=None
      link override convert: arith_type=Boolean  n_bits=1  bin_pt=0
  sampling_frequency_mhz : Subsystem  Tag=xps:sw_reg  AncestorBlock=xps_library/software register  mask(swreg){mode=one value, io_dir=To Processor, io_delay=0, sample_period=1, names=reg, bitwidths=32, arith_types=0, bin_pts=0, sim_port=on, show_format=off}
      mask prompts: io_dir "I/O direction"; io_delay "I/O delay"; sample_period "Sample period"; names "Name:"; bitwidths "Bitwidth:"; arith_types "Type (ufix=0, fix=1, bool=2):"; bin_pts "Binary pt:"; sim_port "Provide sim input/output?"; show_format "Print format string?"
      mask init:
      | swreg_init(gcb)
      settings: AttributesFormatString=1output
      mask TypeOptions mode: one value | fields of equal size | fields of arbitrary size
      mask Callback mode: swreg_cb(gcb);
      mask TypeOptions io_dir: To Processor | From Processor
      mask Callback io_dir:
      | mask_enables = get_param(gcb, 'MaskEnables');
      | mask_names = get_param(gcb, 'MaskNames');
      | if strcmp(get_param(gcb, 'io_dir'), 'To Processor'),
      |     mask_enables{ismember(mask_names, 'sample_period')} = 'off';
      | else
      |     mask_enables{ismember(mask_names, 'sample_period')} = 'on';
      | end
      | set_param(gcb, 'MaskEnables', mask_enables);
      mask Callback bitwidths: swreg_maskcheck(gcb);
      mask Callback arith_types: [numios, ~, ~, ~, current_types] = swreg_maskcheck(gcb);
      mask Callback bin_pts: swreg_maskcheck(gcb);
  stokes : Subsystem
  stokes_enable : Subsystem  Tag=xps:sw_reg  AncestorBlock=xps_library/software register  mask(swreg){mode=one value, io_dir=From Processor, io_delay=0, sample_period=1, names=reg, bitwidths=32, arith_types=0, bin_pts=0, sim_port=on, show_format=off}
      mask prompts: io_dir "I/O direction"; io_delay "I/O delay"; sample_period "Sample period"; names "Name:"; bitwidths "Bitwidth:"; arith_types "Type (ufix=0, fix=1, bool=2):"; bin_pts "Binary pt:"; sim_port "Provide sim input/output?"; show_format "Print format string?"
      mask init:
      | swreg_init(gcb)
      settings: AttributesFormatString=1input
      mask TypeOptions mode: one value | fields of equal size | fields of arbitrary size
      mask Callback mode: swreg_cb(gcb);
      mask TypeOptions io_dir: To Processor | From Processor
      mask Callback io_dir:
      | mask_enables = get_param(gcb, 'MaskEnables');
      | mask_names = get_param(gcb, 'MaskNames');
      | if strcmp(get_param(gcb, 'io_dir'), 'To Processor'),
      |     mask_enables{ismember(mask_names, 'sample_period')} = 'off';
      | else
      |     mask_enables{ismember(mask_names, 'sample_period')} = 'on';
      | end
      | set_param(gcb, 'MaskEnables', mask_enables);
      mask Callback bitwidths:
      | swreg_maskcheck(gcb);
      | % blk = gcb;
      | % mode = get_param(blk, 'mode');
      | % current_widths = eval(get_param(blk, 'bitwidths'));
      | % if (strcmp(mode, 'one value') || strcmp(mode, 'fields of equal size')) && (length(current_widths) > 1),
      | %     error('Only one width may be specified for this mode.');
      | % elseif strcmp(mode, 'fields of arbitrary size')
      | %     current_names = textscan(strtrim(strrep(strrep(get_param(blk, 'names'), ']', ''), '[', '')), '%s');
      | %     current_names = current_names{1};
      | %     numios = length(current_names);
      | %     if length(current_widths) ~= numios,
      | %         error('%d field names specified, but %d widths?', numios, length(current_widths));
      | %     end
      | % end
      | % total_width = 0;
      | % for ctr = 1 : length(current_widths),
      | %     total_width = total_width + current_widths(ctr);
      | % end
      | % if total_width > 32,
      | %     error('Total width must be 32 or less, set to %d.', total_width);
      | % end
      mask Callback arith_types:
      | [numios, ~, ~, ~, current_types] = swreg_maskcheck(gcb);
      | % blk = gcb;
      | % mode = get_param(blk, 'mode');
      | % current_types = eval(get_param(blk, 'arith_types'));
      | % numios = length(current_types);
      | % if (strcmp(mode, 'one value') || strcmp(mode, 'fields of equal size')) && (length(current_types) > 1),
      | %     error('Only one type may be specified for this mode.');
      | % elseif strcmp(mode, 'fields of arbitrary size')
      | %     current_names = textscan(strtrim(strrep(strrep(get_param(blk, 'names'), ']', ''), '[', '')), '%s');
      | %     current_names = current_names{1};
      | %     numios = length(current_names);
      | %     if length(current_types) ~= numios,
      | %         error('%d field names specified, but %d types?', numios, length(current_types));
      | %     end
      | % end
      | problem = 0;
      | for ctr = 1 : numios,
      |     t = current_types(ctr);
      |     if (t < 0) || (t > 2),
      |         problem = t;
      |         ctr = numios + 1;
      |     end
      | end
      | if problem ~= 0,
      |     error('Type cannot be %i, must be 0, 1 or 2.', problem);
      | end
      mask Callback bin_pts:
      | swreg_maskcheck(gcb);
      | % blk = gcb;
      | % mode = get_param(blk, 'mode');
      | % current_bins = eval(get_param(blk, 'bin_pts'));
      | % if (strcmp(mode, 'one value') || strcmp(mode, 'fields of equal size')) && (length(current_bins) > 1),
      | %     error('Only one binary pt may be specified for this mode.');
      | % elseif strcmp(mode, 'fields of arbitrary size')
      | %     current_names = textscan(strtrim(strrep(strrep(get_param(blk, 'names'), ']', ''), '[', '')), '%s');
      | %     current_names = current_names{1};
      | %     numios = length(current_names);
      | %     if length(current_bins) ~= numios,
      | %         error('%d field names specified, but %d binary pts?', numios, length(current_bins));
      | %     end
      | % end
  sub_frame_cnt : xbsIndex_r4/Counter  cnt_type=Free Running  cnt_to=Inf  operation=Up  start_count=0  cnt_by_val=1  arith_type=Unsigned  n_bits=8  bin_pt=0  load_pin=off  rst=on  en=on  explicit_period=on  period=1  dbl_ovrd=off  use_behavioral_HDL=off  implementation=Fabric  block_type=counter
      settings: block_version=11.4
  sync_next_pps : Subsystem  Tag=xps:sw_reg  AncestorBlock=xps_library/software register  DataTypeOverride=Double  DataTypeOverrideAppliesTo=Fixed-point  MinMaxOverflowLogging=ForceOff  mask(swreg){mode=one value, io_dir=From Processor, io_delay=0, sample_period=1, names=reg, bitwidths=32, arith_types=0, bin_pts=[0], sim_port=on, show_format=off}
      mask prompts: io_dir "I/O direction"; io_delay "I/O delay"; sample_period "Sample period"; names "Name:"; bitwidths "Bitwidth:"; arith_types "Type (ufix=0, fix=1, bool=2):"; bin_pts "Binary pt:"; sim_port "Provide sim input/output?"; show_format "Print format string?"
      mask init:
      | swreg_init(gcb)
      settings: AttributesFormatString=1input
      mask TypeOptions mode: one value | fields of equal size | fields of arbitrary size
      mask Callback mode: swreg_cb(gcb);
      mask TypeOptions io_dir: To Processor | From Processor
      mask Callback io_dir:
      | mask_enables = get_param(gcb, 'MaskEnables');
      | mask_names = get_param(gcb, 'MaskNames');
      | if strcmp(get_param(gcb, 'io_dir'), 'To Processor'),
      |     mask_enables{ismember(mask_names, 'sample_period')} = 'off';
      | else
      |     mask_enables{ismember(mask_names, 'sample_period')} = 'on';
      | end
      | set_param(gcb, 'MaskEnables', mask_enables);
      mask Callback bitwidths:
      | swreg_maskcheck(gcb);
      | % blk = gcb;
      | % mode = get_param(blk, 'mode');
      | % current_widths = eval(get_param(blk, 'bitwidths'));
      | % if (strcmp(mode, 'one value') || strcmp(mode, 'fields of equal size')) && (length(current_widths) > 1),
      | %     error('Only one width may be specified for this mode.');
      | % elseif strcmp(mode, 'fields of arbitrary size')
      | %     current_names = textscan(strtrim(strrep(strrep(get_param(blk, 'names'), ']', ''), '[', '')), '%s');
      | %     current_names = current_names{1};
      | %     numios = length(current_names);
      | %     if length(current_widths) ~= numios,
      | %         error('%d field names specified, but %d widths?', numios, length(current_widths));
      | %     end
      | % end
      | % total_width = 0;
      | % for ctr = 1 : length(current_widths),
      | %     total_width = total_width + current_widths(ctr);
      | % end
      | % if total_width > 32,
      | %     error('Total width must be 32 or less, set to %d.', total_width);
      | % end
      mask Callback arith_types:
      | [numios, ~, ~, ~, current_types] = swreg_maskcheck(gcb);
      | % blk = gcb;
      | % mode = get_param(blk, 'mode');
      | % current_types = eval(get_param(blk, 'arith_types'));
      | % numios = length(current_types);
      | % if (strcmp(mode, 'one value') || strcmp(mode, 'fields of equal size')) && (length(current_types) > 1),
      | %     error('Only one type may be specified for this mode.');
      | % elseif strcmp(mode, 'fields of arbitrary size')
      | %     current_names = textscan(strtrim(strrep(strrep(get_param(blk, 'names'), ']', ''), '[', '')), '%s');
      | %     current_names = current_names{1};
      | %     numios = length(current_names);
      | %     if length(current_types) ~= numios,
      | %         error('%d field names specified, but %d types?', numios, length(current_types));
      | %     end
      | % end
      | problem = 0;
      | for ctr = 1 : numios,
      |     t = current_types(ctr);
      |     if (t < 0) || (t > 2),
      |         problem = t;
      |         ctr = numios + 1;
      |     end
      | end
      | if problem ~= 0,
      |     error('Type cannot be %i, must be 0, 1 or 2.', problem);
      | end
      mask Callback bin_pts:
      | swreg_maskcheck(gcb);
      | % blk = gcb;
      | % mode = get_param(blk, 'mode');
      | % current_bins = eval(get_param(blk, 'bin_pts'));
      | % if (strcmp(mode, 'one value') || strcmp(mode, 'fields of equal size')) && (length(current_bins) > 1),
      | %     error('Only one binary pt may be specified for this mode.');
      | % elseif strcmp(mode, 'fields of arbitrary size')
      | %     current_names = textscan(strtrim(strrep(strrep(get_param(blk, 'names'), ']', ''), '[', '')), '%s');
      | %     current_names = current_names{1};
      | %     numios = length(current_names);
      | %     if length(current_bins) ~= numios,
      | %         error('%d field names specified, but %d binary pts?', numios, length(current_bins));
      | %     end
      | % end
  tgbe0 : Subsystem  Tag=xps:tengbe_v2  AncestorBlock=xps_library/ten_Gbe_v2  mask(ten_GbE_v2){flavour=cx4, slot=1, port_r1=2, port_r2_cx4=0, port_r2_sfpp=0, rx_dist_ram=on, large_frames=off, show_param=on, pre_emph_r2=0.74, pre_emph=3, post_emph_r2=0.18, rxeqmix_r2=7, swing_r2=940, swing=800, fab_en=on, fab_mac=hex2dec('123456780000'), fab_ip=10*(2^24) + 0*(2^16) + 0*(2^8) + 2*(2^0), fab_udp=60001, fab_gate=1, cpu_rx_en=on, cpu_tx_en=on, ttl=hex2dec('FF'), promisc_mode=off, debug_ctr_width=16, txctr=on, txerrctr=off, txerrctr_len=4224, txofctr=on, txfullctr=off, txvldctr=on, txsnaplen=8192, rxctr=off, rxerrctr=off, rxerrctr_len=100, rxofctr=off, rxbadctr=off, rxvldctr=off, rxeofctr=off, rxsnaplen=0 - no snap}
      mask prompts: flavour "Mezzanine card flavour"; slot "Card slot"; port_r1 "Port"; port_r2_cx4 "Port"; port_r2_sfpp "Port"; rx_dist_ram "Shallow RX Fifo (Beware overruns!)"; large_frames "Enable Large TX Frames (8k+512)"; show_param "---------------------- Show Implementation Parameters -----------------------------------------------------------------------------------"; pre_emph_r2 "Pre-emphasis (dB)"; pre_emph "Pre-emphasis"; post_emph_r2 "Post-emphasis (dB)"; rxeqmix_r2 "Receive equalisation"; swing_r2 "Driver Swing Control (mVppd)"; swing "Differential swing"; fab_en "Enable fabric on startup"; fab_mac "Fabric MAC Address"; fab_ip "Fabric IP Address"; fab_udp "Fabric UDP Port"; fab_gate "Fabric Gateway"; cpu_rx_en "Enable CPU RX"; cpu_tx_en "Enable CPU TX"; promisc_mode "Promiscuous mode"; debug_ctr_width "Debug counter width"; txctr "TX - core_txctr"; txerrctr "TX packet length error - core_txerrctr"; txerrctr_len "-- expected TX packet length"; txofctr "TX overflow - core_txofctr"; txfullctr "TX full - core_txfullctr"; txvldctr "TX valid cycle - core_txvldctr"; txsnaplen "TX snapshot length"; rxctr "RX - core_rxctr"; rxerrctr "RX packet length error - core_rxerrctr"; rxerrctr_len "-- expected RX packet length"; rxofctr "RX overflow - core_rxofctr"; rxbadctr "RX bad - core_rxbadctr"; rxvldctr "RX valid cycle - core_rxvldctr"; rxeofctr "RX eof - core_rxeofctr"; rxsnaplen "RX snapshot length"
      mask help: This block sends and receives UDP frames (packets). It accepts a 64 bit wide data stream with user-determined frame breaks. The data stream is wrapped in a UDP frame for transmission. Incoming UDP packets are unwrapped and the data presented as a 64 bit wide stream.
      mask init:
      | temp = eval(get_param(gcb, 'debug_ctr_width'));
      | if temp <= 0,
      |     error('Debug counters cannot be ltoet zero.');
      | end
      | tengbe_v2_mask(gcb)
      mask TypeOptions flavour: sfp+ | cx4
      mask Callback flavour: tengbe_v2_callback
      mask TypeOptions slot: 0 | 1
      mask TypeOptions port_r1: 0 | 1 | 2 | 3
      mask TypeOptions port_r2_cx4: 0 | 1 | 2
      mask TypeOptions port_r2_sfpp: 0 | 1 | 2 | 3
      mask Callback show_param: tengbe_v2_callback
      mask TypeOptions pre_emph_r2: 0.15 | 0.3 | 0.45 | 0.61 | 0.74 | 0.91 | 1.07 | 1.25 | 1.36 | 1.55 | 1.74 | 1.94 | 2.11 | 2.32 | 2.54 | 2.77
      mask TypeOptions pre_emph: 0 | 1 | 2 | 3
      mask TypeOptions post_emph_r2: 0.18 | 0.19 | 0.2 | 0.39 | 0.63 | 0.82 | 1.07 | 1.32 | 1.6 | 1.65 | 1.94 | 2.21 | 2.52 | 2.76 | 3.08 | 3.41 | 3.77 | 3.97 | 4.36 | 4.73 | 5.16 | 5.47 | 5.93 | 6.38 | 6.89
      mask TypeOptions rxeqmix_r2: 0 | 1 | 2 | 3 | 4 | 5 | 6 | 7
      mask TypeOptions swing_r2: 110 | 210 | 310 | 400 | 480 | 570 | 660 | 740 | 810 | 880 | 940 | 990 | 1040 | 1080 | 1110 | 1130
      mask TypeOptions swing: 400 | 500 | 600 | 700 | 800
      mask Callback txerrctr:
      | blk = gcb;
      | mask_visibilities = get_param(blk, 'MaskVisibilities');
      | mask_names = get_param(blk, 'MaskNames');
      | if strcmp(get_param(blk, 'txerrctr'), 'on')
      |     mask_visibilities{ismember(mask_names, 'txerrctr_len')} = 'on';
      | else
      |     mask_visibilities{ismember(mask_names, 'txerrctr_len')} = 'off';
      | end
      | set_param(blk, 'MaskVisibilities', mask_visibilities);
      mask TypeOptions txsnaplen: 0 - no snap | 256 | 512 | 1024 | 2048 | 4096 | 8192 | 16384
      mask Callback rxerrctr:
      | blk = gcb;
      | mask_visibilities = get_param(blk, 'MaskVisibilities');
      | mask_names = get_param(blk, 'MaskNames');
      | if strcmp(get_param(blk, 'rxerrctr'), 'on')
      |     mask_visibilities{ismember(mask_names, 'rxerrctr_len')} = 'on';
      | else
      |     mask_visibilities{ismember(mask_names, 'rxerrctr_len')} = 'off';
      | end
      | set_param(blk, 'MaskVisibilities', mask_visibilities);
      mask TypeOptions rxsnaplen: 0 - no snap | 256 | 512 | 1024 | 2048 | 4096 | 8192 | 16384
  tgbe0_debug_reset : Subsystem  Tag=xps:sw_reg  AncestorBlock=xps_library/software register  mask(swreg){mode=one value, io_dir=From Processor, io_delay=0, sample_period=1, names=reg, bitwidths=32, arith_types=0, bin_pts=0, sim_port=on, show_format=off}
      mask prompts: io_dir "I/O direction"; io_delay "I/O delay"; sample_period "Sample period"; names "Name:"; bitwidths "Bitwidth:"; arith_types "Type (ufix=0, fix=1, bool=2):"; bin_pts "Binary pt:"; sim_port "Provide sim input/output?"; show_format "Print format string?"
      mask init:
      | swreg_init(gcb)
      settings: AttributesFormatString=1input
      mask TypeOptions mode: one value | fields of equal size | fields of arbitrary size
      mask Callback mode: swreg_cb(gcb);
      mask TypeOptions io_dir: To Processor | From Processor
      mask Callback io_dir:
      | mask_enables = get_param(gcb, 'MaskEnables');
      | mask_names = get_param(gcb, 'MaskNames');
      | if strcmp(get_param(gcb, 'io_dir'), 'To Processor'),
      |     mask_enables{ismember(mask_names, 'sample_period')} = 'off';
      | else
      |     mask_enables{ismember(mask_names, 'sample_period')} = 'on';
      | end
      | set_param(gcb, 'MaskEnables', mask_enables);
      mask Callback bitwidths: swreg_maskcheck(gcb);
      mask Callback arith_types: [numios, ~, ~, ~, current_types] = swreg_maskcheck(gcb);
      mask Callback bin_pts: swreg_maskcheck(gcb);
  tgbe0_dest_ip : Subsystem  Tag=xps:sw_reg  AncestorBlock=xps_library/software register  mask(swreg){mode=one value, io_dir=From Processor, io_delay=0, sample_period=1, names=reg, bitwidths=32, arith_types=0, bin_pts=0, sim_port=on, show_format=off}
      mask prompts: io_dir "I/O direction"; io_delay "I/O delay"; sample_period "Sample period"; names "Name:"; bitwidths "Bitwidth:"; arith_types "Type (ufix=0, fix=1, bool=2):"; bin_pts "Binary pt:"; sim_port "Provide sim input/output?"; show_format "Print format string?"
      mask init:
      | swreg_init(gcb)
      settings: AttributesFormatString=1input
      mask TypeOptions mode: one value | fields of equal size | fields of arbitrary size
      mask Callback mode: swreg_cb(gcb);
      mask TypeOptions io_dir: To Processor | From Processor
      mask Callback io_dir:
      | mask_enables = get_param(gcb, 'MaskEnables');
      | mask_names = get_param(gcb, 'MaskNames');
      | if strcmp(get_param(gcb, 'io_dir'), 'To Processor'),
      |     mask_enables{ismember(mask_names, 'sample_period')} = 'off';
      | else
      |     mask_enables{ismember(mask_names, 'sample_period')} = 'on';
      | end
      | set_param(gcb, 'MaskEnables', mask_enables);
      mask Callback bitwidths: swreg_maskcheck(gcb);
      mask Callback arith_types: [numios, ~, ~, ~, current_types] = swreg_maskcheck(gcb);
      mask Callback bin_pts: swreg_maskcheck(gcb);
  tgbe0_dest_port : Subsystem  Tag=xps:sw_reg  AncestorBlock=xps_library/software register  mask(swreg){mode=one value, io_dir=From Processor, io_delay=0, sample_period=1, names=reg, bitwidths=16, arith_types=0, bin_pts=0, sim_port=on, show_format=off}
      mask prompts: io_dir "I/O direction"; io_delay "I/O delay"; sample_period "Sample period"; names "Name:"; bitwidths "Bitwidth:"; arith_types "Type (ufix=0, fix=1, bool=2):"; bin_pts "Binary pt:"; sim_port "Provide sim input/output?"; show_format "Print format string?"
      mask init:
      | swreg_init(gcb)
      settings: AttributesFormatString=1input
      mask TypeOptions mode: one value | fields of equal size | fields of arbitrary size
      mask Callback mode: swreg_cb(gcb);
      mask TypeOptions io_dir: To Processor | From Processor
      mask Callback io_dir:
      | mask_enables = get_param(gcb, 'MaskEnables');
      | mask_names = get_param(gcb, 'MaskNames');
      | if strcmp(get_param(gcb, 'io_dir'), 'To Processor'),
      |     mask_enables{ismember(mask_names, 'sample_period')} = 'off';
      | else
      |     mask_enables{ismember(mask_names, 'sample_period')} = 'on';
      | end
      | set_param(gcb, 'MaskEnables', mask_enables);
      mask Callback bitwidths: swreg_maskcheck(gcb);
      mask Callback arith_types: [numios, ~, ~, ~, current_types] = swreg_maskcheck(gcb);
      mask Callback bin_pts: swreg_maskcheck(gcb);
  tgbe0_linkup : Subsystem  Tag=xps:sw_reg  AncestorBlock=xps_library/software register  mask(swreg){mode=one value, io_dir=To Processor, io_delay=0, sample_period=1, names=reg, bitwidths=1, arith_types=2, bin_pts=0, sim_port=on, show_format=off}
      mask prompts: io_dir "I/O direction"; io_delay "I/O delay"; sample_period "Sample period"; names "Name:"; bitwidths "Bitwidth:"; arith_types "Type (ufix=0, fix=1, bool=2):"; bin_pts "Binary pt:"; sim_port "Provide sim input/output?"; show_format "Print format string?"
      mask init:
      | swreg_init(gcb)
      settings: AttributesFormatString=1output
      mask TypeOptions mode: one value | fields of equal size | fields of arbitrary size
      mask Callback mode: swreg_cb(gcb);
      mask TypeOptions io_dir: To Processor | From Processor
      mask Callback io_dir:
      | mask_enables = get_param(gcb, 'MaskEnables');
      | mask_names = get_param(gcb, 'MaskNames');
      | if strcmp(get_param(gcb, 'io_dir'), 'To Processor'),
      |     mask_enables{ismember(mask_names, 'sample_period')} = 'off';
      | else
      |     mask_enables{ismember(mask_names, 'sample_period')} = 'on';
      | end
      | set_param(gcb, 'MaskEnables', mask_enables);
      mask Callback bitwidths:
      | swreg_maskcheck(gcb);
      | % blk = gcb;
      | % mode = get_param(blk, 'mode');
      | % current_widths = eval(get_param(blk, 'bitwidths'));
      | % if (strcmp(mode, 'one value') || strcmp(mode, 'fields of equal size')) && (length(current_widths) > 1),
      | %     error('Only one width may be specified for this mode.');
      | % elseif strcmp(mode, 'fields of arbitrary size')
      | %     current_names = textscan(strtrim(strrep(strrep(get_param(blk, 'names'), ']', ''), '[', '')), '%s');
      | %     current_names = current_names{1};
      | %     numios = length(current_names);
      | %     if length(current_widths) ~= numios,
      | %         error('%d field names specified, but %d widths?', numios, length(current_widths));
      | %     end
      | % end
      | % total_width = 0;
      | % for ctr = 1 : length(current_widths),
      | %     total_width = total_width + current_widths(ctr);
      | % end
      | % if total_width > 32,
      | %     error('Total width must be 32 or less, set to %d.', total_width);
      | % end
      mask Callback arith_types:
      | [numios, ~, ~, ~, current_types] = swreg_maskcheck(gcb);
      | % blk = gcb;
      | % mode = get_param(blk, 'mode');
      | % current_types = eval(get_param(blk, 'arith_types'));
      | % numios = length(current_types);
      | % if (strcmp(mode, 'one value') || strcmp(mode, 'fields of equal size')) && (length(current_types) > 1),
      | %     error('Only one type may be specified for this mode.');
      | % elseif strcmp(mode, 'fields of arbitrary size')
      | %     current_names = textscan(strtrim(strrep(strrep(get_param(blk, 'names'), ']', ''), '[', '')), '%s');
      | %     current_names = current_names{1};
      | %     numios = length(current_names);
      | %     if length(current_types) ~= numios,
      | %         error('%d field names specified, but %d types?', numios, length(current_types));
      | %     end
      | % end
      | problem = 0;
      | for ctr = 1 : numios,
      |     t = current_types(ctr);
      |     if (t < 0) || (t > 2),
      |         problem = t;
      |         ctr = numios + 1;
      |     end
      | end
      | if problem ~= 0,
      |     error('Type cannot be %i, must be 0, 1 or 2.', problem);
      | end
      mask Callback bin_pts:
      | swreg_maskcheck(gcb);
      | % blk = gcb;
      | % mode = get_param(blk, 'mode');
      | % current_bins = eval(get_param(blk, 'bin_pts'));
      | % if (strcmp(mode, 'one value') || strcmp(mode, 'fields of equal size')) && (length(current_bins) > 1),
      | %     error('Only one binary pt may be specified for this mode.');
      | % elseif strcmp(mode, 'fields of arbitrary size')
      | %     current_names = textscan(strtrim(strrep(strrep(get_param(blk, 'names'), ']', ''), '[', '')), '%s');
      | %     current_names = current_names{1};
      | %     numios = length(current_names);
      | %     if length(current_bins) ~= numios,
      | %         error('%d field names specified, but %d binary pts?', numios, length(current_bins));
      | %     end
      | % end
  tgbe0_tx : Subsystem  Tag=xps:sw_reg  AncestorBlock=xps_library/software register  mask(swreg){mode=one value, io_dir=To Processor, io_delay=0, sample_period=1, names=reg, bitwidths=1, arith_types=2, bin_pts=0, sim_port=on, show_format=off}
      mask prompts: io_dir "I/O direction"; io_delay "I/O delay"; sample_period "Sample period"; names "Name:"; bitwidths "Bitwidth:"; arith_types "Type (ufix=0, fix=1, bool=2):"; bin_pts "Binary pt:"; sim_port "Provide sim input/output?"; show_format "Print format string?"
      mask init:
      | swreg_init(gcb)
      settings: AttributesFormatString=1output
      mask TypeOptions mode: one value | fields of equal size | fields of arbitrary size
      mask Callback mode: swreg_cb(gcb);
      mask TypeOptions io_dir: To Processor | From Processor
      mask Callback io_dir:
      | mask_enables = get_param(gcb, 'MaskEnables');
      | mask_names = get_param(gcb, 'MaskNames');
      | if strcmp(get_param(gcb, 'io_dir'), 'To Processor'),
      |     mask_enables{ismember(mask_names, 'sample_period')} = 'off';
      | else
      |     mask_enables{ismember(mask_names, 'sample_period')} = 'on';
      | end
      | set_param(gcb, 'MaskEnables', mask_enables);
      mask Callback bitwidths:
      | swreg_maskcheck(gcb);
      | % blk = gcb;
      | % mode = get_param(blk, 'mode');
      | % current_widths = eval(get_param(blk, 'bitwidths'));
      | % if (strcmp(mode, 'one value') || strcmp(mode, 'fields of equal size')) && (length(current_widths) > 1),
      | %     error('Only one width may be specified for this mode.');
      | % elseif strcmp(mode, 'fields of arbitrary size')
      | %     current_names = textscan(strtrim(strrep(strrep(get_param(blk, 'names'), ']', ''), '[', '')), '%s');
      | %     current_names = current_names{1};
      | %     numios = length(current_names);
      | %     if length(current_widths) ~= numios,
      | %         error('%d field names specified, but %d widths?', numios, length(current_widths));
      | %     end
      | % end
      | % total_width = 0;
      | % for ctr = 1 : length(current_widths),
      | %     total_width = total_width + current_widths(ctr);
      | % end
      | % if total_width > 32,
      | %     error('Total width must be 32 or less, set to %d.', total_width);
      | % end
      mask Callback arith_types:
      | [numios, ~, ~, ~, current_types] = swreg_maskcheck(gcb);
      | % blk = gcb;
      | % mode = get_param(blk, 'mode');
      | % current_types = eval(get_param(blk, 'arith_types'));
      | % numios = length(current_types);
      | % if (strcmp(mode, 'one value') || strcmp(mode, 'fields of equal size')) && (length(current_types) > 1),
      | %     error('Only one type may be specified for this mode.');
      | % elseif strcmp(mode, 'fields of arbitrary size')
      | %     current_names = textscan(strtrim(strrep(strrep(get_param(blk, 'names'), ']', ''), '[', '')), '%s');
      | %     current_names = current_names{1};
      | %     numios = length(current_names);
      | %     if length(current_types) ~= numios,
      | %         error('%d field names specified, but %d types?', numios, length(current_types));
      | %     end
      | % end
      | problem = 0;
      | for ctr = 1 : numios,
      |     t = current_types(ctr);
      |     if (t < 0) || (t > 2),
      |         problem = t;
      |         ctr = numios + 1;
      |     end
      | end
      | if problem ~= 0,
      |     error('Type cannot be %i, must be 0, 1 or 2.', problem);
      | end
      mask Callback bin_pts:
      | swreg_maskcheck(gcb);
      | % blk = gcb;
      | % mode = get_param(blk, 'mode');
      | % current_bins = eval(get_param(blk, 'bin_pts'));
      | % if (strcmp(mode, 'one value') || strcmp(mode, 'fields of equal size')) && (length(current_bins) > 1),
      | %     error('Only one binary pt may be specified for this mode.');
      | % elseif strcmp(mode, 'fields of arbitrary size')
      | %     current_names = textscan(strtrim(strrep(strrep(get_param(blk, 'names'), ']', ''), '[', '')), '%s');
      | %     current_names = current_names{1};
      | %     numios = length(current_names);
      | %     if length(current_bins) ~= numios,
      | %         error('%d field names specified, but %d binary pts?', numios, length(current_bins));
      | %     end
      | % end
  tgbe0_tx_full : Subsystem  Tag=xps:sw_reg  AncestorBlock=xps_library/software register  mask(swreg){mode=one value, io_dir=To Processor, io_delay=0, sample_period=1, names=reg, bitwidths=1, arith_types=2, bin_pts=0, sim_port=on, show_format=off}
      mask prompts: io_dir "I/O direction"; io_delay "I/O delay"; sample_period "Sample period"; names "Name:"; bitwidths "Bitwidth:"; arith_types "Type (ufix=0, fix=1, bool=2):"; bin_pts "Binary pt:"; sim_port "Provide sim input/output?"; show_format "Print format string?"
      mask init:
      | swreg_init(gcb)
      settings: AttributesFormatString=1output
      mask TypeOptions mode: one value | fields of equal size | fields of arbitrary size
      mask Callback mode: swreg_cb(gcb);
      mask TypeOptions io_dir: To Processor | From Processor
      mask Callback io_dir:
      | mask_enables = get_param(gcb, 'MaskEnables');
      | mask_names = get_param(gcb, 'MaskNames');
      | if strcmp(get_param(gcb, 'io_dir'), 'To Processor'),
      |     mask_enables{ismember(mask_names, 'sample_period')} = 'off';
      | else
      |     mask_enables{ismember(mask_names, 'sample_period')} = 'on';
      | end
      | set_param(gcb, 'MaskEnables', mask_enables);
      mask Callback bitwidths:
      | swreg_maskcheck(gcb);
      | % blk = gcb;
      | % mode = get_param(blk, 'mode');
      | % current_widths = eval(get_param(blk, 'bitwidths'));
      | % if (strcmp(mode, 'one value') || strcmp(mode, 'fields of equal size')) && (length(current_widths) > 1),
      | %     error('Only one width may be specified for this mode.');
      | % elseif strcmp(mode, 'fields of arbitrary size')
      | %     current_names = textscan(strtrim(strrep(strrep(get_param(blk, 'names'), ']', ''), '[', '')), '%s');
      | %     current_names = current_names{1};
      | %     numios = length(current_names);
      | %     if length(current_widths) ~= numios,
      | %         error('%d field names specified, but %d widths?', numios, length(current_widths));
      | %     end
      | % end
      | % total_width = 0;
      | % for ctr = 1 : length(current_widths),
      | %     total_width = total_width + current_widths(ctr);
      | % end
      | % if total_width > 32,
      | %     error('Total width must be 32 or less, set to %d.', total_width);
      | % end
      mask Callback arith_types:
      | [numios, ~, ~, ~, current_types] = swreg_maskcheck(gcb);
      | % blk = gcb;
      | % mode = get_param(blk, 'mode');
      | % current_types = eval(get_param(blk, 'arith_types'));
      | % numios = length(current_types);
      | % if (strcmp(mode, 'one value') || strcmp(mode, 'fields of equal size')) && (length(current_types) > 1),
      | %     error('Only one type may be specified for this mode.');
      | % elseif strcmp(mode, 'fields of arbitrary size')
      | %     current_names = textscan(strtrim(strrep(strrep(get_param(blk, 'names'), ']', ''), '[', '')), '%s');
      | %     current_names = current_names{1};
      | %     numios = length(current_names);
      | %     if length(current_types) ~= numios,
      | %         error('%d field names specified, but %d types?', numios, length(current_types));
      | %     end
      | % end
      | problem = 0;
      | for ctr = 1 : numios,
      |     t = current_types(ctr);
      |     if (t < 0) || (t > 2),
      |         problem = t;
      |         ctr = numios + 1;
      |     end
      | end
      | if problem ~= 0,
      |     error('Type cannot be %i, must be 0, 1 or 2.', problem);
      | end
      mask Callback bin_pts:
      | swreg_maskcheck(gcb);
      | % blk = gcb;
      | % mode = get_param(blk, 'mode');
      | % current_bins = eval(get_param(blk, 'bin_pts'));
      | % if (strcmp(mode, 'one value') || strcmp(mode, 'fields of equal size')) && (length(current_bins) > 1),
      | %     error('Only one binary pt may be specified for this mode.');
      | % elseif strcmp(mode, 'fields of arbitrary size')
      | %     current_names = textscan(strtrim(strrep(strrep(get_param(blk, 'names'), ']', ''), '[', '')), '%s');
      | %     current_names = current_names{1};
      | %     numios = length(current_names);
      | %     if length(current_bins) ~= numios,
      | %         error('%d field names specified, but %d binary pts?', numios, length(current_bins));
      | %     end
      | % end
  tgbe0_tx_of : Subsystem  Tag=xps:sw_reg  AncestorBlock=xps_library/software register  mask(swreg){mode=one value, io_dir=To Processor, io_delay=0, sample_period=1, names=reg, bitwidths=1, arith_types=2, bin_pts=0, sim_port=on, show_format=off}
      mask prompts: io_dir "I/O direction"; io_delay "I/O delay"; sample_period "Sample period"; names "Name:"; bitwidths "Bitwidth:"; arith_types "Type (ufix=0, fix=1, bool=2):"; bin_pts "Binary pt:"; sim_port "Provide sim input/output?"; show_format "Print format string?"
      mask init:
      | swreg_init(gcb)
      settings: AttributesFormatString=1output
      mask TypeOptions mode: one value | fields of equal size | fields of arbitrary size
      mask Callback mode: swreg_cb(gcb);
      mask TypeOptions io_dir: To Processor | From Processor
      mask Callback io_dir:
      | mask_enables = get_param(gcb, 'MaskEnables');
      | mask_names = get_param(gcb, 'MaskNames');
      | if strcmp(get_param(gcb, 'io_dir'), 'To Processor'),
      |     mask_enables{ismember(mask_names, 'sample_period')} = 'off';
      | else
      |     mask_enables{ismember(mask_names, 'sample_period')} = 'on';
      | end
      | set_param(gcb, 'MaskEnables', mask_enables);
      mask Callback bitwidths:
      | swreg_maskcheck(gcb);
      | % blk = gcb;
      | % mode = get_param(blk, 'mode');
      | % current_widths = eval(get_param(blk, 'bitwidths'));
      | % if (strcmp(mode, 'one value') || strcmp(mode, 'fields of equal size')) && (length(current_widths) > 1),
      | %     error('Only one width may be specified for this mode.');
      | % elseif strcmp(mode, 'fields of arbitrary size')
      | %     current_names = textscan(strtrim(strrep(strrep(get_param(blk, 'names'), ']', ''), '[', '')), '%s');
      | %     current_names = current_names{1};
      | %     numios = length(current_names);
      | %     if length(current_widths) ~= numios,
      | %         error('%d field names specified, but %d widths?', numios, length(current_widths));
      | %     end
      | % end
      | % total_width = 0;
      | % for ctr = 1 : length(current_widths),
      | %     total_width = total_width + current_widths(ctr);
      | % end
      | % if total_width > 32,
      | %     error('Total width must be 32 or less, set to %d.', total_width);
      | % end
      mask Callback arith_types:
      | [numios, ~, ~, ~, current_types] = swreg_maskcheck(gcb);
      | % blk = gcb;
      | % mode = get_param(blk, 'mode');
      | % current_types = eval(get_param(blk, 'arith_types'));
      | % numios = length(current_types);
      | % if (strcmp(mode, 'one value') || strcmp(mode, 'fields of equal size')) && (length(current_types) > 1),
      | %     error('Only one type may be specified for this mode.');
      | % elseif strcmp(mode, 'fields of arbitrary size')
      | %     current_names = textscan(strtrim(strrep(strrep(get_param(blk, 'names'), ']', ''), '[', '')), '%s');
      | %     current_names = current_names{1};
      | %     numios = length(current_names);
      | %     if length(current_types) ~= numios,
      | %         error('%d field names specified, but %d types?', numios, length(current_types));
      | %     end
      | % end
      | problem = 0;
      | for ctr = 1 : numios,
      |     t = current_types(ctr);
      |     if (t < 0) || (t > 2),
      |         problem = t;
      |         ctr = numios + 1;
      |     end
      | end
      | if problem ~= 0,
      |     error('Type cannot be %i, must be 0, 1 or 2.', problem);
      | end
      mask Callback bin_pts:
      | swreg_maskcheck(gcb);
      | % blk = gcb;
      | % mode = get_param(blk, 'mode');
      | % current_bins = eval(get_param(blk, 'bin_pts'));
      | % if (strcmp(mode, 'one value') || strcmp(mode, 'fields of equal size')) && (length(current_bins) > 1),
      | %     error('Only one binary pt may be specified for this mode.');
      | % elseif strcmp(mode, 'fields of arbitrary size')
      | %     current_names = textscan(strtrim(strrep(strrep(get_param(blk, 'names'), ']', ''), '[', '')), '%s');
      | %     current_names = current_names{1};
      | %     numios = length(current_names);
      | %     if length(current_bins) ~= numios,
      | %         error('%d field names specified, but %d binary pts?', numios, length(current_bins));
      | %     end
      | % end
  time_lsb : Subsystem  Tag=xps:sw_reg  AncestorBlock=xps_library/software register  DataTypeOverride=Double  DataTypeOverrideAppliesTo=Fixed-point  MinMaxOverflowLogging=ForceOff  mask(swreg){mode=one value, io_dir=From Processor, io_delay=0, sample_period=1, names=reg, bitwidths=32, arith_types=0, bin_pts=[0], sim_port=on, show_format=off}
      mask prompts: io_dir "I/O direction"; io_delay "I/O delay"; sample_period "Sample period"; names "Name:"; bitwidths "Bitwidth:"; arith_types "Type (ufix=0, fix=1, bool=2):"; bin_pts "Binary pt:"; sim_port "Provide sim input/output?"; show_format "Print format string?"
      mask init:
      | swreg_init(gcb)
      settings: AttributesFormatString=1input
      mask TypeOptions mode: one value | fields of equal size | fields of arbitrary size
      mask Callback mode: swreg_cb(gcb);
      mask TypeOptions io_dir: To Processor | From Processor
      mask Callback io_dir:
      | mask_enables = get_param(gcb, 'MaskEnables');
      | mask_names = get_param(gcb, 'MaskNames');
      | if strcmp(get_param(gcb, 'io_dir'), 'To Processor'),
      |     mask_enables{ismember(mask_names, 'sample_period')} = 'off';
      | else
      |     mask_enables{ismember(mask_names, 'sample_period')} = 'on';
      | end
      | set_param(gcb, 'MaskEnables', mask_enables);
      mask Callback bitwidths:
      | swreg_maskcheck(gcb);
      | % blk = gcb;
      | % mode = get_param(blk, 'mode');
      | % current_widths = eval(get_param(blk, 'bitwidths'));
      | % if (strcmp(mode, 'one value') || strcmp(mode, 'fields of equal size')) && (length(current_widths) > 1),
      | %     error('Only one width may be specified for this mode.');
      | % elseif strcmp(mode, 'fields of arbitrary size')
      | %     current_names = textscan(strtrim(strrep(strrep(get_param(blk, 'names'), ']', ''), '[', '')), '%s');
      | %     current_names = current_names{1};
      | %     numios = length(current_names);
      | %     if length(current_widths) ~= numios,
      | %         error('%d field names specified, but %d widths?', numios, length(current_widths));
      | %     end
      | % end
      | % total_width = 0;
      | % for ctr = 1 : length(current_widths),
      | %     total_width = total_width + current_widths(ctr);
      | % end
      | % if total_width > 32,
      | %     error('Total width must be 32 or less, set to %d.', total_width);
      | % end
      mask Callback arith_types:
      | [numios, ~, ~, ~, current_types] = swreg_maskcheck(gcb);
      | % blk = gcb;
      | % mode = get_param(blk, 'mode');
      | % current_types = eval(get_param(blk, 'arith_types'));
      | % numios = length(current_types);
      | % if (strcmp(mode, 'one value') || strcmp(mode, 'fields of equal size')) && (length(current_types) > 1),
      | %     error('Only one type may be specified for this mode.');
      | % elseif strcmp(mode, 'fields of arbitrary size')
      | %     current_names = textscan(strtrim(strrep(strrep(get_param(blk, 'names'), ']', ''), '[', '')), '%s');
      | %     current_names = current_names{1};
      | %     numios = length(current_names);
      | %     if length(current_types) ~= numios,
      | %         error('%d field names specified, but %d types?', numios, length(current_types));
      | %     end
      | % end
      | problem = 0;
      | for ctr = 1 : numios,
      |     t = current_types(ctr);
      |     if (t < 0) || (t > 2),
      |         problem = t;
      |         ctr = numios + 1;
      |     end
      | end
      | if problem ~= 0,
      |     error('Type cannot be %i, must be 0, 1 or 2.', problem);
      | end
      mask Callback bin_pts:
      | swreg_maskcheck(gcb);
      | % blk = gcb;
      | % mode = get_param(blk, 'mode');
      | % current_bins = eval(get_param(blk, 'bin_pts'));
      | % if (strcmp(mode, 'one value') || strcmp(mode, 'fields of equal size')) && (length(current_bins) > 1),
      | %     error('Only one binary pt may be specified for this mode.');
      | % elseif strcmp(mode, 'fields of arbitrary size')
      | %     current_names = textscan(strtrim(strrep(strrep(get_param(blk, 'names'), ']', ''), '[', '')), '%s');
      | %     current_names = current_names{1};
      | %     numios = length(current_names);
      | %     if length(current_bins) ~= numios,
      | %         error('%d field names specified, but %d binary pts?', numios, length(current_bins));
      | %     end
      | % end
  time_msb : Subsystem  Tag=xps:sw_reg  AncestorBlock=xps_library/software register  DataTypeOverride=Double  DataTypeOverrideAppliesTo=Fixed-point  MinMaxOverflowLogging=ForceOff  mask(swreg){mode=one value, io_dir=From Processor, io_delay=0, sample_period=1, names=reg, bitwidths=32, arith_types=0, bin_pts=[0], sim_port=on, show_format=off}
      mask prompts: io_dir "I/O direction"; io_delay "I/O delay"; sample_period "Sample period"; names "Name:"; bitwidths "Bitwidth:"; arith_types "Type (ufix=0, fix=1, bool=2):"; bin_pts "Binary pt:"; sim_port "Provide sim input/output?"; show_format "Print format string?"
      mask init:
      | swreg_init(gcb)
      settings: AttributesFormatString=1input
      mask TypeOptions mode: one value | fields of equal size | fields of arbitrary size
      mask Callback mode: swreg_cb(gcb);
      mask TypeOptions io_dir: To Processor | From Processor
      mask Callback io_dir:
      | mask_enables = get_param(gcb, 'MaskEnables');
      | mask_names = get_param(gcb, 'MaskNames');
      | if strcmp(get_param(gcb, 'io_dir'), 'To Processor'),
      |     mask_enables{ismember(mask_names, 'sample_period')} = 'off';
      | else
      |     mask_enables{ismember(mask_names, 'sample_period')} = 'on';
      | end
      | set_param(gcb, 'MaskEnables', mask_enables);
      mask Callback bitwidths:
      | swreg_maskcheck(gcb);
      | % blk = gcb;
      | % mode = get_param(blk, 'mode');
      | % current_widths = eval(get_param(blk, 'bitwidths'));
      | % if (strcmp(mode, 'one value') || strcmp(mode, 'fields of equal size')) && (length(current_widths) > 1),
      | %     error('Only one width may be specified for this mode.');
      | % elseif strcmp(mode, 'fields of arbitrary size')
      | %     current_names = textscan(strtrim(strrep(strrep(get_param(blk, 'names'), ']', ''), '[', '')), '%s');
      | %     current_names = current_names{1};
      | %     numios = length(current_names);
      | %     if length(current_widths) ~= numios,
      | %         error('%d field names specified, but %d widths?', numios, length(current_widths));
      | %     end
      | % end
      | % total_width = 0;
      | % for ctr = 1 : length(current_widths),
      | %     total_width = total_width + current_widths(ctr);
      | % end
      | % if total_width > 32,
      | %     error('Total width must be 32 or less, set to %d.', total_width);
      | % end
      mask Callback arith_types:
      | [numios, ~, ~, ~, current_types] = swreg_maskcheck(gcb);
      | % blk = gcb;
      | % mode = get_param(blk, 'mode');
      | % current_types = eval(get_param(blk, 'arith_types'));
      | % numios = length(current_types);
      | % if (strcmp(mode, 'one value') || strcmp(mode, 'fields of equal size')) && (length(current_types) > 1),
      | %     error('Only one type may be specified for this mode.');
      | % elseif strcmp(mode, 'fields of arbitrary size')
      | %     current_names = textscan(strtrim(strrep(strrep(get_param(blk, 'names'), ']', ''), '[', '')), '%s');
      | %     current_names = current_names{1};
      | %     numios = length(current_names);
      | %     if length(current_types) ~= numios,
      | %         error('%d field names specified, but %d types?', numios, length(current_types));
      | %     end
      | % end
      | problem = 0;
      | for ctr = 1 : numios,
      |     t = current_types(ctr);
      |     if (t < 0) || (t > 2),
      |         problem = t;
      |         ctr = numios + 1;
      |     end
      | end
      | if problem ~= 0,
      |     error('Type cannot be %i, must be 0, 1 or 2.', problem);
      | end
      mask Callback bin_pts:
      | swreg_maskcheck(gcb);
      | % blk = gcb;
      | % mode = get_param(blk, 'mode');
      | % current_bins = eval(get_param(blk, 'bin_pts'));
      | % if (strcmp(mode, 'one value') || strcmp(mode, 'fields of equal size')) && (length(current_bins) > 1),
      | %     error('Only one binary pt may be specified for this mode.');
      | % elseif strcmp(mode, 'fields of arbitrary size')
      | %     current_names = textscan(strtrim(strrep(strrep(get_param(blk, 'names'), ']', ''), '[', '')), '%s');
      | %     current_names = current_names{1};
      | %     numios = length(current_names);
      | %     if length(current_bins) ~= numios,
      | %         error('%d field names specified, but %d binary pts?', numios, length(current_bins));
      | %     end
      | % end
  upper_adc_threshold : Subsystem  Tag=xps:sw_reg  AncestorBlock=xps_library/software register  DataTypeOverride=Double  DataTypeOverrideAppliesTo=Fixed-point  MinMaxOverflowLogging=ForceOff  mask(swreg){mode=one value, io_dir=From Processor, io_delay=0, sample_period=1, names=reg, bitwidths=32, arith_types=0, bin_pts=[0], sim_port=off, show_format=off}
      mask prompts: io_dir "I/O direction"; io_delay "I/O delay"; sample_period "Sample period"; names "Name:"; bitwidths "Bitwidth:"; arith_types "Type (ufix=0, fix=1, bool=2):"; bin_pts "Binary pt:"; sim_port "Provide sim input/output?"; show_format "Print format string?"
      mask init:
      | swreg_init(gcb)
      settings: AttributesFormatString=1input
      mask TypeOptions mode: one value | fields of equal size | fields of arbitrary size
      mask Callback mode: swreg_cb(gcb);
      mask TypeOptions io_dir: To Processor | From Processor
      mask Callback io_dir:
      | mask_enables = get_param(gcb, 'MaskEnables');
      | mask_names = get_param(gcb, 'MaskNames');
      | if strcmp(get_param(gcb, 'io_dir'), 'To Processor'),
      |     mask_enables{ismember(mask_names, 'sample_period')} = 'off';
      | else
      |     mask_enables{ismember(mask_names, 'sample_period')} = 'on';
      | end
      | set_param(gcb, 'MaskEnables', mask_enables);
      mask Callback bitwidths:
      | swreg_maskcheck(gcb);
      | % blk = gcb;
      | % mode = get_param(blk, 'mode');
      | % current_widths = eval(get_param(blk, 'bitwidths'));
      | % if (strcmp(mode, 'one value') || strcmp(mode, 'fields of equal size')) && (length(current_widths) > 1),
      | %     error('Only one width may be specified for this mode.');
      | % elseif strcmp(mode, 'fields of arbitrary size')
      | %     current_names = textscan(strtrim(strrep(strrep(get_param(blk, 'names'), ']', ''), '[', '')), '%s');
      | %     current_names = current_names{1};
      | %     numios = length(current_names);
      | %     if length(current_widths) ~= numios,
      | %         error('%d field names specified, but %d widths?', numios, length(current_widths));
      | %     end
      | % end
      | % total_width = 0;
      | % for ctr = 1 : length(current_widths),
      | %     total_width = total_width + current_widths(ctr);
      | % end
      | % if total_width > 32,
      | %     error('Total width must be 32 or less, set to %d.', total_width);
      | % end
      mask Callback arith_types:
      | [numios, ~, ~, ~, current_types] = swreg_maskcheck(gcb);
      | % blk = gcb;
      | % mode = get_param(blk, 'mode');
      | % current_types = eval(get_param(blk, 'arith_types'));
      | % numios = length(current_types);
      | % if (strcmp(mode, 'one value') || strcmp(mode, 'fields of equal size')) && (length(current_types) > 1),
      | %     error('Only one type may be specified for this mode.');
      | % elseif strcmp(mode, 'fields of arbitrary size')
      | %     current_names = textscan(strtrim(strrep(strrep(get_param(blk, 'names'), ']', ''), '[', '')), '%s');
      | %     current_names = current_names{1};
      | %     numios = length(current_names);
      | %     if length(current_types) ~= numios,
      | %         error('%d field names specified, but %d types?', numios, length(current_types));
      | %     end
      | % end
      | problem = 0;
      | for ctr = 1 : numios,
      |     t = current_types(ctr);
      |     if (t < 0) || (t > 2),
      |         problem = t;
      |         ctr = numios + 1;
      |     end
      | end
      | if problem ~= 0,
      |     error('Type cannot be %i, must be 0, 1 or 2.', problem);
      | end
      mask Callback bin_pts:
      | swreg_maskcheck(gcb);
      | % blk = gcb;
      | % mode = get_param(blk, 'mode');
      | % current_bins = eval(get_param(blk, 'bin_pts'));
      | % if (strcmp(mode, 'one value') || strcmp(mode, 'fields of equal size')) && (length(current_bins) > 1),
      | %     error('Only one binary pt may be specified for this mode.');
      | % elseif strcmp(mode, 'fields of arbitrary size')
      | %     current_names = textscan(strtrim(strrep(strrep(get_param(blk, 'names'), ']', ''), '[', '')), '%s');
      | %     current_names = current_names{1};
      | %     numios = length(current_names);
      | %     if length(current_bins) ~= numios,
      | %         error('%d field names specified, but %d binary pts?', numios, length(current_bins));
      | %     end
      | % end
  window_size1 : xbsIndex_r4/Constant  const=200  gui_display_data_type=Fixed-point  arith_type=Unsigned  n_bits=32  bin_pt=0  preci_type=Single  exp_width=8  frac_width=24  explicit_period=off  period=1  equ=P=C  opselect=C  inp2=PCIN>>17  opr=+  inp1=P  carry=CIN  dbl_ovrd=off  block_type=constant
  xsg_core_config : xps_library/XSG core config  Tag=xps:xsg  hw_sys=ROACH:sx95t  clk_src=adc0_clk  ROACH_clk_src=adc0_clk  ROACH2_clk_src=sys_clk  MKDIG_clk_src=sys_clk  clk_rate=200  sample_period=1  synthesis_tool=XST
  wires:
  Band-Limited White Noise/1 -> Sum/2
  Sine Wave/1 -> Sum/1
  Pulse Generator/1 -> katadc/3(sim_sync)
  Constant5/1 -> katadc/4(sim_data_valid)
  Sum/1 -> katadc/2(sim_data1), katadc/1(sim_data0)
  katadc/11(sync0) -> Delay189/1
  katadc/12(sync1) -> Delay190/1
  katadc/13(sync2) -> Delay191/1
  katadc/14(sync3) -> Delay192/1
  pfb_fir_real/1(sync_out) -> Delay84/1
  coarse_fft_shift_mask/1(in_reg) -> Delay15/1
  Constant6/1 -> coarse_fft_shift_mask/1(sim_1)
  err_clear_sim4/1 -> tgbe0_dest_port/1(sim_1)
  tgbe0_dest_port/1(in_reg) -> Delay38/1
  err_clear_sim3/1 -> tgbe0_dest_ip/1(sim_1)
  tgbe0_dest_ip/1(in_reg) -> Delay37/1
  packetizer/3(data_valid) -> [packetiser_dout_v]
  Constant9/1 -> tgbe0/7(rx_ack), tgbe0/8(rx_overrun_ack)
  tgbe0/6(rx_data) -> Terminator5/1
  tgbe0/7(rx_valid) -> Terminator6/1
  tgbe0/8(rx_source_ip) -> Terminator7/1
  tgbe0/9(rx_source_port) -> Terminator8/1
  tgbe0/10(rx_end_of_frame) -> Terminator9/1
  tgbe0/11(rx_bad_frame) -> Terminator10/1
  posedge1/1(out) -> Logical8/1, [eth_eof]
  accumulation_length/1(in_reg) -> Delay36/1
  accumlation_count/1 -> accumulation_length/1(sim_1)
  Constant1/1 -> adc0_en/1(sim_1)
  Constant3/1 -> adc0_atten/1(sim_1)
  adc1_en/1(in_reg) -> Slice32/1
  adc0_en/1(in_reg) -> Slice30/1
  Logical3/1 -> Counter2/1
  Concat2/1 -> Delay28/1
  Relational1/1 -> Logical3/1, posedge/1(in)
  tgbe0/1(led_up) -> [eth_up], Delay32/1
  tgbe0/2(led_rx) -> Terminator20/1
  tgbe0/3(led_tx) -> Delay31/1
  Delay11/1 -> tgbe0_tx_of/1(out_reg)
  Delay30/1 -> tgbe0_tx_full/1(out_reg)
  Delay31/1 -> tgbe0_tx/1(out_reg)
  Delay32/1 -> tgbe0_linkup/1(out_reg)
  Delay33/1 -> tgbe0/1(rst)
  accumulation_cnt/1(sim_out) -> Terminator1/1
  Delay34/1 -> Slice1/1, accumulation_cnt/1(out_reg)
  Delay35/1 -> fft_wideband_real/2(shift)
  Delay37/1 -> tgbe0/4(tx_dest_ip)
  Delay38/1 -> tgbe0/5(tx_dest_port)
  Counter3/1 -> Delay8/1, Delay40/1
  eth_eof_cnt/1(sim_out) -> Terminator3/1
  Delay40/1 -> eth_eof_cnt/1(out_reg)
  Delay41/1 -> Counter3/2
  Counter2/1 -> Relational1/1, Delay34/1
  Signal Builder/1(Signal 1) -> eth_reset/1(sim_1)
  eth_reset/1(in_reg) -> Slice/1
  [eth_reset] -> Delay53/1
  Delay53/1 -> Counter3/1
  Delay56/1 -> pfb_fir_real/1(sync)
  Delay28/1 -> packetizer/2(din)
  manual_sync/1(in_reg) -> Slice2/1
  Constant8/1 -> manual_sync/1(sim_1)
  Slice2/1 -> posedge5/1(in)
  acc_trig_cnt/1(sim_out) -> Terminator30/1
  Counter10/1 -> acc_trig_cnt/1(out_reg)
  posedge10/1(out) -> Counter10/1
  [acc_trig] -> posedge10/1(in)
  Counter11/1 -> [packet_length_cnt], Relational2/1
  Logical8/1 -> Counter11/1
  [queue_empty] -> Inverter2/1
  Mux/1 -> [eth_tx_data], tgbe0/2(tx_data)
  Logical20/1 -> Delay49/1
  packetizer/4(buffer_overflow) -> [packetiser_of]
  [packetiser_din_v] -> posedge11/1(in)
  [eth_reset] -> posedge13/1(in)
  Logical9/1 -> Counter12/1
  posedge12/1(out) -> Counter12/2
  Delay29/1 -> packetizer/1(din_valid)
  Counter12/1 -> Slice6/1
  Slice6/1 -> Logical10/1
  Logical10/1 -> Delay177/1
  Inverter/1 -> Logical9/2
  tgbe0_linkup/1(sim_out) -> Terminator2/1
  tgbe0_tx/1(sim_out) -> Terminator4/1
  tgbe0_tx_full/1(sim_out) -> Terminator11/1
  tgbe0_tx_of/1(sim_out) -> Terminator17/1
  Delay68/1 -> Inverter/1, Logical10/2, posedge12/1(in)
  packetiser_of_cnt/1(sim_out) -> Terminator18/1
  Delay74/1 -> packetiser_of_cnt/1(out_reg)
  posedge13/1(out) -> Delay33/1
  err_clear_sim1/1 -> tgbe0_debug_reset/1(sim_1)
  tgbe0_debug_reset/1(in_reg) -> Delay78/1
  Delay78/1 -> Slice7/1
  Slice7/1 -> tgbe0/9(debug_rst)
  tgbe0/12(rx_overrun) -> Terminator19/1
  Delay84/1 -> fft_wideband_real/1(sync), [pfb_sync_out]
  Delay85/1 -> fft_wideband_real/3(in00)
  Delay86/1 -> fft_wideband_real/4(in01)
  Delay88/1 -> fft_wideband_real/5(in02)
  Delay89/1 -> fft_wideband_real/6(in03)
  Delay90/1 -> fft_wideband_real1/3(in00)
  Delay91/1 -> fft_wideband_real1/4(in01)
  Delay92/1 -> fft_wideband_real1/5(in02)
  Delay93/1 -> fft_wideband_real1/6(in03)
  packetiser_perc_full/1(sim_out) -> Terminator12/1
  [packetiser_perc_full] -> Delay104/1
  Delay104/1 -> packetiser_perc_full/1(out_reg)
  packetizer/2(data_sout) -> [packetiser_dout]
  packetizer/1(data_addr) -> [packetiser_addr]
  [packetiser_dout_v] -> Delay113/1
  [packetiser_dout] -> Delay112/1
  Delay112/1 -> FIFO/1
  Delay113/1 -> FIFO/2
  Delay114/1 -> FIFO/4
  [eth_reset] -> Delay114/1
  [eth_eof] -> Delay94/1
  [eth_eof] -> Delay41/1
  [eth_data_tx_valid] -> FIFO/3
  FIFO/2 -> [queue_empty]
  [eth_reset] -> Logical8/2
  FIFO/4 -> [queue_full]
  FIFO/1 -> [queue_dout]
  Counter13/1 -> [interpacket_length_cnt], Relational4/1
  Logical11/1 -> Counter13/1
  Delay116/1 -> Slice16/1
  Relational4/1 -> posedge14/1(in)
  [eth_reset] -> Logical11/2
  eth_interframe_length_/1 -> eth_interpacket_length/1(sim_1)
  eth_interpacket_length/1(in_reg) -> Delay116/1
  Logical12/1 -> Counter11/2, [eth_data_tx_valid]
  Counter14/1 -> Slice13/1
  [eth_eof] -> Logical13/1
  Logical13/1 -> Counter14/2
  [hdr_send_end] -> Logical13/2
  [eth_eof] -> Logical14/1
  Logical14/1 -> Counter15/2
  [interpacket_end] -> Logical14/2
  Relational2/1 -> posedge1/1(in)
  [eth_reset] -> Counter14/1
  posedge14/1(out) -> Logical11/1, [interpacket_end]
  [eth_reset] -> Counter15/1
  Counter15/1 -> Slice14/1
  FIFO/3 -> [queue_perc_full]
  Slice13/1 -> Logical12/2
  Slice14/1 -> [interpacket_valid], Counter13/2
  tgbe0/4(tx_afull) -> Delay30/1
  Delay94/1 -> tgbe0/6(tx_end_of_frame)
  queue_perc_full/1(sim_out) -> Terminator21/1
  [queue_perc_full] -> Delay124/1
  Delay124/1 -> queue_perc_full/1(out_reg)
  queue_empty/1(sim_out) -> Terminator24/1
  [queue_empty] -> Delay125/1
  Delay125/1 -> queue_empty/1(out_reg)
  eth_packet_length_cnt/1(sim_out) -> Terminator25/1
  [packet_length_cnt] -> Delay126/1
  Delay126/1 -> eth_packet_length_cnt/1(out_reg)
  eth_interpacket_length_cnt/1(sim_out) -> Terminator26/1
  [interpacket_length_cnt] -> Delay127/1
  Delay127/1 -> eth_interpacket_length_cnt/1(out_reg)
  Logical15/1 -> Delay68/1
  Slice/1 -> Logical15/1
  [fine_pfb0_sync_out] -> Delay51/1
  Delay51/1 -> Logical15/2
  Counter6/1 -> Delay74/1
  [packetiser_of] -> Delay57/1
  posedge15/1(out) -> Counter6/2
  Delay57/1 -> posedge15/1(in)
  [eth_reset] -> Delay58/1
  Delay58/1 -> Counter6/1
  packetizer/5(perc_full) -> [packetiser_perc_full]
  Delay52/1 -> packetizer/3(reset)
  [eth_reset] -> Delay52/1
  packetizer/6(done) -> [packetiser_done]
  Counter16/1 -> [hdr_length_cnt], Relational5/1
  Logical18/1 -> Counter16/1
  hdr_size/1 -> Relational5/2
  Relational5/1 -> posedge8/1(in)
  [eth_reset] -> Logical18/2
  [interpacket_end] -> Logical19/1
  Logical19/1 -> Counter17/2
  [hdr_send_end] -> Logical19/2
  posedge8/1(out) -> Logical18/1, [hdr_send_end]
  [eth_reset] -> Counter17/1
  Counter17/1 -> Slice8/1
  Slice8/1 -> Logical17/1, Counter16/2
  magic_no/1 -> Concat4/1
  [eth_reset] -> Delay144/1
  sub_frame_cnt/1 -> Relational6/1, [hdr_subframe_cnt], Concat4/3
  Logical21/1 -> sub_frame_cnt/1
  Delay144/1 -> Logical21/2
  [eth_eof] -> sub_frame_cnt/2
  Concat4/1 -> [hdr_dout]
  posedge11/1(out) -> Logical9/1
  Delay141/1 -> Mux/2
  [hdr_dout] -> Slice10/1, Slice9/1
  Delay140/1 -> Mux/3
  Slice9/1 -> Delay141/1
  Slice10/1 -> Delay140/1
  [queue_dout] -> Delay3/1
  Concat5/1 -> [eth_mux_select], Delay142/1
  [eth_hdr_tx_valid] -> Logical22/1, Inverter3/1
  Relational6/1 -> Logical21/1
  [eth_reset] -> Inverter1/1
  Inverter1/1 -> Logical17/2
  Logical17/1 -> [eth_hdr_tx_valid]
  Delay142/1 -> Mux/1
  Inverter3/1 -> Concat5/1
  [hdr_length_cnt] -> Slice11/1
  Logical22/1 -> Concat5/2
  Slice11/1 -> Logical22/2
  Inverter2/1 -> Logical12/1
  [eth_hdr_tx_valid] -> Logical20/2
  Delay49/1 -> tgbe0/3(tx_valid)
  [eth_data_tx_valid] -> Logical20/1
  Delay3/1 -> Mux/4
  Delay5/1 -> Slice17/1
  eth_interframe_length_1/1 -> eth_packets_per_accum_window/1(sim_1)
  eth_packets_per_accum_window/1(in_reg) -> Delay5/1
  "1 "/1 -> AddSub/2
  Slice16/1 -> Relational4/2
  [eth_packets_per_accum_window] -> Delay170/1
  Slice17/1 -> [eth_packets_per_accum_window]
  Delay170/1 -> Concat4/4
  Shift/1 -> AddSub/1
  Delay171/1 -> Slice19/1
  eth_interframe_length_2/1 -> eth_data_size_per_packet/1(sim_1)
  eth_data_size_per_packet/1(in_reg) -> Delay171/1
  Slice19/1 -> [eth_data_size_per_packet]
  posedge/1(out) -> Delay151/1
  eth_cycles_per_packet/1(sim_out) -> Terminator16/1
  Delay50/1 -> eth_cycles_per_packet/1(out_reg)
  AddSub/1 -> Delay48/1
  sync_next_pps/1(in_reg) -> Slice18/1
  Signal Builder1/1(Signal 1) -> sync_next_pps/1(sim_1)
  posedge16/1(out) -> Delay168/1
  Slice18/1 -> posedge16/1(in)
  Delay168/1 -> [sync_next_pps], Counter18/2
  Logical16/1 -> [sync_pulse]
  [sync_pulse] -> Delay56/1
  Counter18/1 -> Slice15/1
  Delay172/1 -> Counter18/1
  roach_led0/1 -> Terminator27/1
  roach_led1/1 -> Terminator31/1
  roach_led2/1 -> Terminator32/1
  roach_led3/1 -> Terminator33/1
  roach_led4/1 -> Terminator37/1
  roach_led5/1 -> Terminator34/1
  roach_led6/1 -> Terminator36/1
  roach_led7/1 -> Terminator35/1
  tgbe0/5(tx_overflow) -> [eth_tx_of], Delay11/1
  [eth_data_size_per_packet] -> Shift/1
  Delay48/1 -> Delay50/1, Relational2/2
  Logical23/1 -> Logical16/1
  Delay77/1 -> Logical16/2
  [sync_pulse] -> Delay172/1
  posedge5/1(out) -> Delay77/1
  Delay8/1 -> Slice12/1
  Slice12/1 -> [eth_eof_led]
  Slice1/1 -> [acc_trig_led]
  roach_sma_j10/1 -> Terminator38/1
  Delay108/1 -> roach_sma_j10/1
  Logical27/1 -> [noise_diode_on], Delay108/1
  err_clear_sim2/1 -> noise_diode_en/1(sim_1)
  noise_diode_en/1(in_reg) -> Slice4/1
  Slice4/1 -> Delay107/1, [noise_diode_enable]
  Counter20/1 -> [noise_diode_on_cnt], Relational8/1
  Logical28/1 -> Counter20/1
  Delay111/1 -> Relational8/2
  Relational8/1 -> posedge6/1(in)
  [noise_diode_on_end] -> Logical29/1
  Logical29/1 -> Counter21/2
  [noise_diode_off_end] -> Logical29/2
  posedge6/1(out) -> Logical28/1, [noise_diode_on_end]
  Logical33/1 -> Counter21/1, Logical28/2
  Counter21/1 -> Slice23/1
  Slice23/1 -> Logical31/1, Inverter5/1, [noise_diode_duty_cycle_on]
  err_clear_sim5/1 -> noise_diode_on_length/1(sim_1)
  noise_diode_on_length/1(in_reg) -> Delay111/1
  Counter4/1 -> [noise_diode_off_cnt], Relational7/1
  Logical25/1 -> Counter4/1
  Delay109/1 -> Relational7/2
  Relational7/1 -> posedge4/1(in)
  [eth_reset] -> Logical25/2
  [noise_diode_on_end] -> Logical26/1
  Logical26/1 -> Counter5/2
  [noise_diode_off_end] -> Logical26/2
  posedge4/1(out) -> Logical25/1, [noise_diode_off_end]
  [eth_reset] -> Counter5/1
  Counter5/1 -> Slice22/1
  Slice22/1 -> Logical30/1, [noise_diode_duty_cycle_off]
  err_clear_sim6/1 -> noise_diode_off_length/1(sim_1)
  noise_diode_off_length/1(in_reg) -> Delay109/1
  [noise_diode_duty_cycle_on] -> Delay146/1
  Logical30/1 -> Counter4/2
  [acc_trig] -> Logical30/2
  Logical31/1 -> Counter20/2
  [acc_trig] -> Delay123/1
  Logical32/1 -> Logical29/3
  Inverter5/1 -> Logical32/4
  [noise_diode_enable] -> Logical32/2
  [noise_diode_enable] -> posedge17/1(in)
  posedge17/1(out) -> Logical33/1
  [eth_reset] -> Logical33/2
  hdr_size2/1 -> Delay120/1, Delay121/1
  roach_gpio_a_enable_not/1 -> Terminator39/1
  roach_gpio_b_enable_not/1 -> Terminator40/1
  Delay120/1 -> roach_gpio_a_enable_not/1
  Delay121/1 -> roach_gpio_b_enable_not/1
  Delay123/1 -> Logical32/1
  err_clear_sim7/1 -> noise_diode_duty_cycle_en/1(sim_1)
  noise_diode_duty_cycle_en/1(in_reg) -> Slice24/1
  Slice24/1 -> Inverter6/1
  Inverter6/1 -> Delay145/1
  Logical34/1 -> Logical27/2
  Delay107/1 -> Logical27/1
  Delay145/1 -> Logical34/1
  Delay146/1 -> Logical34/2
  Delay147/1 -> Counter2/2
  [noise_diode_duty_cycle_off] -> Inverter7/1
  Inverter7/1 -> Logical32/3
  [acc_trig] -> Logical31/2
  Delay151/1 -> [acc_trig]
  katadc/15(data_valid) -> Terminator14/1
  Counter23/1 -> Register19/1
  Register19/1 -> Relational/1, Relational9/1, clk_frequency/1(out_reg)
  clk_frequency/1(sim_out) -> Terminator46/1
  [pps] -> Counter23/1, Register19/2
  Constant10/1 -> Relational/2
  Constant37/1 -> Relational9/2
  Relational/1 -> Logical7/1
  Relational9/1 -> Logical7/2
  Logical7/1 -> [clk_bad]
  [pps] -> Delay60/1
  Delay60/1 -> Counter/1
  Counter/1 -> Slice5/1
  Slice5/1 -> Delay64/1
  Delay64/1 -> roach_led7/1
  [eth_up] -> Delay6/1
  Delay47/1 -> roach_led6/1
  Delay6/1 -> Delay47/1
  Delay65/1 -> roach_led5/1
  [eth_eof_led] -> Delay63/1
  Delay63/1 -> Delay65/1
  Delay67/1 -> roach_led4/1
  [noise_diode_led] -> Delay61/1
  Delay61/1 -> Delay67/1
  Delay39/1 -> roach_led2/1
  Delay44/1 -> roach_led3/1
  Delay66/1 -> roach_led1/1
  [clk_bad] -> Delay46/1
  Delay46/1 -> Delay66/1
  Delay62/1 -> Delay152/1
  [of_led] -> Delay62/1
  Delay152/1 -> roach_led0/1
  Logical24/1 -> [of_led]
  [sync_pulse] -> Logical35/1, Counter22/1
  Constant11/1 -> time_lsb/1(sim_1)
  Counter22/1 -> [rtc]
  Constant12/1 -> time_msb/1(sim_1)
  Concat8/1 -> Reinterpret8/1
  time_msb/1(in_reg) -> Concat8/1
  time_lsb/1(in_reg) -> Concat8/2
  Counter24/1 -> Relational10/1
  window_size1/1 -> Relational10/2
  Relational10/1 -> posedge18/1(in)
  posedge18/1(out) -> Logical38/1, Logical35/2, [usec_tick]
  Counter25/1 -> [dsp_delay_cnt], Register1/1
  Register1/1 -> Delay153/1
  [sync_pulse] -> Counter25/1
  [fine_fft_done] -> Logical37/1
  [wait_for_pps] -> Counter26/1
  [fine_fft_done] -> Logical36/1
  Logical36/1 -> Counter26/2
  Logical37/1 -> Register1/2
  Delay143/1 -> Logical37/2
  [usec_tick] -> Counter25/2
  [rtc] -> Register2/1
  Register2/1 -> Delay154/1
  [acc_trig] -> Register2/2
  dsp_delay/1(sim_out) -> Terminator15/1
  Delay153/1 -> Delay155/1, [dsp_delay]
  Delay155/1 -> dsp_delay/1(out_reg)
  last_timestamp_lsb/1(sim_out) -> Terminator47/1
  Delay156/1 -> last_timestamp_lsb/1(out_reg)
  [dsp_delay] -> AddSub1/2
  Delay154/1 -> AddSub1/1
  last_timestamp_msb/1(sim_out) -> Terminator48/1
  Delay157/1 -> last_timestamp_msb/1(out_reg)
  AddSub1/1 -> Slice27/1, Slice26/1, [timestamp]
  Slice26/1 -> Delay157/1
  Slice27/1 -> Delay156/1
  [timestamp] -> Reinterpret9/1
  Slice15/1 -> [wait_for_pps], Logical23/2
  Reinterpret8/1 -> Counter22/2
  Counter26/1 -> Slice28/1
  Slice28/1 -> Logical36/2, Delay143/1
  Reinterpret9/1 -> Concat4/2
  [wait_for_pps] -> Logical38/2
  Logical38/1 -> Counter24/1
  Delay177/1 -> [eth_reset]
  another1/1 -> AddSub2/2
  [eth_packets_per_accum_window] -> Delay139/1
  AddSub2/1 -> Delay200/1
  Logical35/1 -> Counter22/3
  Delay189/1 -> Logical/1
  Delay190/1 -> Logical/2
  Delay191/1 -> Logical/3
  Delay192/1 -> Logical/4
  Delay193/1 -> katadc/8(atten1)
  Delay194/1 -> katadc/7(en1)
  Delay195/1 -> katadc/6(atten0)
  Delay196/1 -> katadc/5(en0)
  Delay200/1 -> Relational6/2
  fft_wideband_real/1(sync_out) -> Delay206/1
  fft_wideband_real/2(out00) -> Delay205/1
  fft_wideband_real/3(out01) -> Delay203/1
  Delay201/1 -> [coarse_channel_select]
  constant7/1 -> fine_fft0/6, fine_fft0/5
  buffer1/3(d_out) -> Delay81/1
  constant13/1 -> fine_fft1/5, fine_fft1/6
  fine_fft0/1 -> Delay4/1
  coarse_channel_select/1(in_reg) -> Delay201/1
  Constant7/1 -> coarse_channel_select/1(sim_1)
  channel_select_dv_cnt/1(sim_out) -> Terminator44/1
  Counter28/1 -> Delay137/1
  Delay79/1 -> pfb_fir_async/3(pol1_in1)
  Delay136/1 -> Counter28/2
  Delay137/1 -> channel_select_dv_cnt/1(out_reg)
  [sync_pulse] -> Delay138/1
  Delay138/1 -> Counter28/1
  posedge9/1(out) -> Delay136/1
  Mux1/1 -> Delay165/1
  Delay165/1 -> [noise_diode_led]
  [noise_diode_enable] -> Delay213/1
  [noise_diode_on] -> Delay212/1
  Delay213/1 -> Concat1/1
  Delay212/1 -> Concat1/2
  Concat1/1 -> Delay214/1
  Delay214/1 -> Mux1/1
  Constant15/1 -> Delay215/1
  Constant16/1 -> Delay217/1
  Counter30/1 -> Slice33/1
  Relational11/1 -> posedge19/1(in)
  Counter31/1 -> Relational11/1
  Constant17/1 -> Relational11/2
  Delay166/1 -> Counter31/1, Counter30/1
  posedge19/1(out) -> Delay166/1
  [usec_tick] -> Delay167/1
  Delay167/1 -> Counter31/2
  Slice33/1 -> Delay216/1
  Delay215/1 -> Mux1/2, Mux1/3
  Delay217/1 -> Mux1/5
  Delay216/1 -> Mux1/4
  [fine_pfb0_sync_out] -> Logical3/2
  Delay139/1 -> AddSub2/1
  buffer1/2(dv) -> Delay80/1
  buffer0/1(sync_out) -> Delay27/1
  Delay162/1 -> posedge2/1(in), [fine_pfb0_dv_out]
  Delay163/1 -> [fine_pfb0_sync_out]
  Delay197/1 -> [pps]
  posedge3/1(out) -> Delay197/1
  Logical/1 -> posedge3/1(in)
  [pps] -> Logical23/1
  pps_cnt/1(sim_out) -> Terminator23/1
  Counter7/1 -> Delay76/1
  Delay76/1 -> pps_cnt/1(out_reg)
  Delay87/1 -> Counter7/2
  [sync_pulse] -> Counter7/1
  [pps] -> Delay87/1
  overflows/1(sim_out) -> Terminator13/1
  assert/1 -> fine_fft0/4
  assert1/1 -> fine_fft1/4
  Delay233/1 -> Delay128/1
  Delay227/1 -> Delay97/1
  Logical5/1 -> Delay29/1, [packetiser_din_v]
  fine_fft1/9 -> [fine_fft1_done]
  fine_fft0/9 -> [fine_fft0_done]
  fine_fft1/7 -> Delay208/1
  fine_fft0/7 -> Delay150/1
  [fine_fft1_done] -> assert1/1
  [fine_fft0_done] -> assert/1
  posedge2/1(out) -> [fine_pfb0_dv_out_edge]
  [fine_pfb0_dv_out_edge] -> fine_fft0/3
  [fine_pfb1_dv_out_edge] -> fine_fft1/3
  fine_fft0/2 -> Delay131/1
  fine_fft1/2 -> Delay207/1
  fine_fft1/1 -> Delay160/1
  Delay150/1 -> [fine_fft0_dv]
  Delay208/1 -> [fine_fft1_dv]
  [fine_pfb1_sync_out] -> fine_fft1/7
  [fine_pfb0_sync_out] -> fine_fft0/7
  Logical40/1 -> [fine_fft_done]
  [fine_fft0_done] -> Logical40/1
  [fine_fft1_done] -> Logical40/2
  Logical2/1 -> [fine_fft_dv]
  [fine_fft0_dv] -> Logical2/1
  [fine_fft1_dv] -> Logical2/2
  [adc1_or] -> Delay149/1
  Delay149/1 -> pulse_ext/1
  pulse_ext/1 -> overflows/6(out_adc1_or), Logical24/6
  [adc0_or] -> Delay148/1
  Delay148/1 -> pulse_ext1/1
  pulse_ext1/1 -> Logical24/7, overflows/7(out_adc0_or)
  [packetiser_of] -> Delay9/1
  Delay9/1 -> pulse_ext4/1
  [queue_full] -> Delay43/1
  Delay43/1 -> pulse_ext3/1
  [eth_tx_of] -> Delay45/1
  Delay45/1 -> pulse_ext2/1
  pulse_ext2/1 -> overflows/1(out_eth_tx_of), Logical24/1
  pulse_ext3/1 -> overflows/2(out_fifo_full), Logical24/2
  pulse_ext4/1 -> Logical24/3, overflows/3(out_packetiser_of)
  [coarse_fft0_overflow] -> Delay42/1
  Delay42/1 -> pulse_ext6/1
  pulse_ext5/1 -> overflows/5(out_coarse_fft0_of), Logical24/5
  pulse_ext6/1 -> overflows/4(out_coarse_fft1_of), Logical24/4
  [stokes_done_out] -> Delay147/1
  pfb_fir_async/1(sync_out) -> Delay163/1
  pfb_fir_async/2(dv_out) -> Delay162/1
  pfb_fir_async/3(pol1_out1) -> Delay161/1
  Delay115/1 -> stokes/3(left_imag)
  Delay117/1 -> stokes/4(right_real)
  Delay118/1 -> stokes/5(right_imag)
  Delay103/1 -> [fft_done_out], stokes/1(sync_in)
  stokes/3(stokes_q) -> Delay219/1
  stokes/4(stokes_u) -> Delay220/1
  stokes/6(l_power) -> Delay222/1
  stokes/7(r_power) -> Delay223/1
  [fine_fft_dv] -> Delay129/1
  [fine_fft_done] -> Delay130/1
  stokes/10(dv_out) -> Delay224/1
  Delay133/1 -> stokes/6(dv_in)
  stokes/1(sync_out) -> Delay164/1
  Delay164/1 -> [stokes_done_out]
  stokes/2(stokes_i) -> Terminator42/1
  Delay219/1 -> [stokes_q]
  Delay220/1 -> [stokes_u]
  stokes/5(stokes_v) -> Terminator43/1
  Delay222/1 -> [l_power]
  Delay223/1 -> [r_power]
  Delay224/1 -> [stokes_dv_out]
  Delay110/1 -> stokes/2(left_real)
  convert/1(out) -> Delay110/1
  convert1/1(out) -> Delay115/1
  convert2/1(out) -> Delay117/1
  convert3/1(out) -> Delay118/1
  [fine_fft0_r] -> [fine_fft0_r_reint], convert/1(in)
  [fine_fft0_i] -> convert1/1(in)
  [fine_fft1_r] -> convert2/1(in)
  [fine_fft1_i] -> convert3/1(in)
  Delay129/1 -> Delay133/1
  Delay130/1 -> Delay103/1
  Delay203/1 -> [coarse_fft_dout_01]
  Delay205/1 -> [coarse_fft_dout_00]
  Delay206/1 -> [coarse_fft_sync_out]
  [coarse_fft_sync_out] -> buffer0/1(sync_in)
  [coarse_channel_select] -> buffer0/2(chan_sel)
  [coarse_fft_dout_00] -> buffer0/3(data_in_even)
  [coarse_fft_dout_01] -> buffer0/4(data_in_odd)
  [coarse_fft_dout_10] -> buffer1/3(data_in_even)
  [coarse_fft_dout_11] -> buffer1/4(data_in_odd)
  [coarse_fft_sync_out] -> buffer1/1(sync_in)
  [coarse_channel_select] -> buffer1/2(chan_sel)
  async_bram_vacc/2(valid) -> Delay234/1
  async_bram_vacc/1(dout) -> Delay233/1
  [acc_trig] -> Delay158/1
  Delay106/1 -> Delay98/1
  Delay228/1 -> Delay134/1
  Delay158/1 -> Delay102/1
  [l_power] -> Delay228/1
  [stokes_dv_out] -> Delay106/1
  [acc_trig] -> Delay176/1
  Delay173/1 -> Delay105/1
  Delay178/1 -> Delay132/1
  Delay176/1 -> Delay119/1
  [r_power] -> Delay178/1
  [stokes_dv_out] -> Delay173/1
  [acc_trig] -> Delay17/1
  Delay209/1 -> async_bram_vacc2/3(en)
  Delay210/1 -> async_bram_vacc2/2(new_acc)
  [stokes_dv_out] -> Delay18/1
  [acc_trig] -> Delay21/1
  Delay225/1 -> async_bram_vacc3/3(en)
  Delay226/1 -> async_bram_vacc3/2(new_acc)
  [stokes_dv_out] -> Delay23/1
  async_bram_vacc1/1(dout) -> Delay227/1
  async_bram_vacc1/2(valid) -> Delay231/1
  Delay7/1 -> pfb_fir_real1/1(sync)
  [sync_pulse] -> Delay7/1
  pfb_fir_real1/1(sync_out) -> Delay24/1
  Delay22/1 -> fft_wideband_real1/2(shift)
  Delay15/1 -> Delay22/1, Delay35/1
  Delay24/1 -> fft_wideband_real1/1(sync)
  fft_wideband_real1/2(out00) -> Delay204/1
  Delay204/1 -> [coarse_fft_dout_10]
  Delay2/1 -> [coarse_fft1_overflow]
  fft_wideband_real1/3(out01) -> Delay202/1
  fft_wideband_real1/4(of) -> Slice21/1
  Delay202/1 -> [coarse_fft_dout_11]
  fft_wideband_real1/1(sync_out) -> Terminator22/1
  Delay25/1 -> [coarse_fft0_overflow]
  fft_wideband_real/4(of) -> Slice29/1
  buffer1/1(sync_out) -> Delay59/1
  buffer0/2(dv) -> Delay1/1
  buffer0/3(d_out) -> Delay79/1
  Delay27/1 -> pfb_fir_async/1(sync), [fine_pfb_sync_in]
  Delay1/1 -> pfb_fir_async/2(dv), [coarse_fft_buffer_dv], posedge9/1(in)
  Delay59/1 -> pfb_fir_async1/1(sync)
  Delay80/1 -> pfb_fir_async1/2(dv)
  Delay81/1 -> pfb_fir_async1/3(pol1_in1)
  Delay161/1 -> [fine_pfb0_dout]
  [fine_pfb0_dout] -> c_to_ri5/1
  Delay99/1 -> [fine_pfb1_dv_out], posedge7/1(in)
  Delay100/1 -> [fine_pfb1_sync_out]
  posedge7/1(out) -> [fine_pfb1_dv_out_edge]
  pfb_fir_async1/1(sync_out) -> Delay100/1
  pfb_fir_async1/2(dv_out) -> Delay99/1
  pfb_fir_async1/3(pol1_out1) -> Delay83/1
  Delay83/1 -> [fine_pfb1_dout]
  [fine_pfb1_dout] -> c_to_ri4/1
  [coarse_fft1_overflow] -> Delay101/1
  Delay101/1 -> pulse_ext5/1
  Slice21/1 -> Delay2/1
  Slice29/1 -> Delay25/1
  c_to_ri5/1 -> fine_fft0/1
  c_to_ri5/2 -> fine_fft0/2
  c_to_ri4/1 -> fine_fft1/1
  c_to_ri4/2 -> fine_fft1/2
  pfb_fir_real1/5(pol1_out4) -> Delay93/1
  pfb_fir_real1/4(pol1_out3) -> Delay92/1
  pfb_fir_real1/3(pol1_out2) -> Delay91/1
  pfb_fir_real1/2(pol1_out1) -> Delay90/1
  pfb_fir_real/5(pol1_out4) -> Delay89/1
  pfb_fir_real/4(pol1_out3) -> Delay88/1
  pfb_fir_real/3(pol1_out2) -> Delay86/1
  pfb_fir_real/2(pol1_out1) -> Delay85/1
  Delay4/1 -> [fine_fft0_r]
  Delay131/1 -> [fine_fft0_i]
  Delay160/1 -> [fine_fft1_r]
  Delay207/1 -> [fine_fft1_i]
  stokes/8(l_phase) -> Delay10/1
  stokes/9(r_phase) -> Delay12/1
  Delay10/1 -> [l_phase]
  Delay12/1 -> [r_phase]
  Delay234/1 -> Delay229/1
  Delay231/1 -> Delay122/1
  [dvalid_3] -> Logical5/4
  [dvalid_2] -> Logical5/3
  [dvalid_0] -> Logical5/1
  [dvalid_1] -> Logical5/2
  stokes_enable/1(in_reg) -> Slice3/1
  accumlation_count1/1 -> stokes_enable/1(sim_1)
  Slice3/1 -> Delay236/1
  Delay17/1 -> Delay19/1
  Delay18/1 -> Delay20/1
  Delay19/1 -> Delay210/1
  Delay20/1 -> Delay209/1
  Delay13/1 -> async_bram_vacc3/1(din)
  Mux7/1 -> Delay13/1
  Delay236/1 -> [stokes_enable]
  Delay239/1 -> Mux7/1
  [stokes_u] -> Delay14/1
  Delay14/1 -> Mux7/3
  [l_phase] -> Delay16/1
  Delay16/1 -> Mux7/2
  Delay21/1 -> Delay72/1
  Delay23/1 -> Delay73/1
  Delay26/1 -> async_bram_vacc2/1(din)
  Mux2/1 -> Delay26/1
  Delay71/1 -> Mux2/1
  [stokes_q] -> Delay69/1
  Delay69/1 -> Mux2/3
  [r_phase] -> Delay70/1
  Delay70/1 -> Mux2/2
  Delay72/1 -> Delay226/1
  Delay73/1 -> Delay225/1
  [stokes_enable] -> Delay71/1
  [stokes_enable] -> Delay239/1
  Reinterpret3/1 -> Concat2/4
  Reinterpret4/1 -> Concat2/3
  Reinterpret5/1 -> Concat2/2
  Reinterpret7/1 -> Concat2/1
  async_bram_vacc2/2(valid) -> Delay82/1
  async_bram_vacc2/1(dout) -> Delay75/1
  Delay82/1 -> Delay232/1
  async_bram_vacc3/2(valid) -> Delay96/1
  async_bram_vacc3/1(dout) -> Delay95/1
  Delay96/1 -> Delay237/1
  Delay98/1 -> Delay211/1
  Delay102/1 -> Delay135/1
  Delay105/1 -> Delay159/1
  Delay132/1 -> Delay174/1
  Delay119/1 -> Delay169/1
  Delay134/1 -> Delay175/1
  Delay169/1 -> async_bram_vacc1/2(new_acc)
  Delay135/1 -> async_bram_vacc/2(new_acc)
  Delay159/1 -> async_bram_vacc1/3(en)
  Delay174/1 -> async_bram_vacc1/1(din)
  Delay211/1 -> async_bram_vacc/3(en)
  Delay175/1 -> async_bram_vacc/1(din)
  [dout_3] -> Reinterpret3/1
  [dout_2] -> Reinterpret4/1
  [dout_0] -> Reinterpret7/1
  [dout_1] -> Reinterpret5/1
  Delay36/1 -> [acc_length], Relational1/2
  Concat6/1 -> Concat4/5
  [stokes_enable] -> Delay245/1
  [noise_diode_on] -> Concat6/1
  Delay245/1 -> Concat6/3
  another2/1 -> Concat6/2
  pps_cnt1/1(sim_out) -> Terminator28/1
  Constant13/1 -> Delay218/1
  Delay218/1 -> pps_cnt1/1(out_reg)
  sampling_frequency_mhz/1(sim_out) -> Terminator29/1
  Constant14/1 -> Delay221/1
  Delay221/1 -> sampling_frequency_mhz/1(out_reg)
  coarse_fft_size_nsamp/1(sim_out) -> Terminator41/1
  Constant18/1 -> Delay241/1
  Delay241/1 -> coarse_fft_size_nsamp/1(out_reg)
  fine_fft_size_nsamp/1(sim_out) -> Terminator45/1
  Constant19/1 -> Delay242/1
  Delay242/1 -> fine_fft_size_nsamp/1(out_reg)
  adc0_atten/1(in_reg) -> Slice31/1
  adc1_atten/1(in_reg) -> Slice20/1
  accum_samples_per_clk/1(sim_out) -> Terminator51/1
  Constant20/1 -> Delay246/1
  Delay246/1 -> accum_samples_per_clk/1(out_reg)
  Slice20/1 -> Delay193/1
  Slice30/1 -> Delay196/1
  Slice31/1 -> Delay195/1
  Slice32/1 -> Delay194/1
  Constant2/1 -> adc1_en/1(sim_1)
  Constant4/1 -> adc1_atten/1(sim_1)
  Delay95/1 -> Delay235/1
  Delay75/1 -> Delay230/1
  Delay237/1 -> [dvalid_3]
  Delay97/1 -> [dout_1]
  Delay122/1 -> [dvalid_1]
  Delay229/1 -> [dvalid_0]
  Delay235/1 -> [dout_3]
  Delay232/1 -> [dvalid_2]
  Delay128/1 -> [dout_0]
  Delay230/1 -> [dout_2]
  [adc_data0_0] -> Delay262/1
  Delay262/1 -> reinterpret10/1
  Delay269/1 -> Mult3/2, Mult3/1
  Mult3/1 -> Reinterpret12/1
  Delay270/1 -> accumulator/1
  accumulator/1 -> Delay271/1
  relational12/1 -> Delay292/1
  relational13/1 -> Delay290/1
  Register3/1 -> Delay283/1, relational12/1, relational13/1
  counter27/1 -> relational14/1
  relational14/1 -> posedge20/1(in)
  posedge20/1(out) -> counter27/1, Delay275/1
  adc_threshold_acc_length/1(in_reg) -> Delay274/1
  upper_adc_threshold/1(in_reg) -> Delay272/1
  lower_adc_threshold/1(in_reg) -> Delay273/1
  Delay272/1 -> [adc_upper_threshold]
  Delay273/1 -> [adc_lower_threshold]
  Delay274/1 -> relational14/2
  Delay275/1 -> [adc_threshold_acc_trig]
  [adc_lower_threshold] -> relational13/2
  [adc_upper_threshold] -> relational12/2
  [adc_data1_0] -> Delay266/1
  Delay266/1 -> reinterpret11/1
  Delay280/1 -> Mult1/1, Mult1/2
  Mult1/1 -> Reinterpret13/1
  Delay281/1 -> accumulator1/1
  accumulator1/1 -> Delay282/1
  relational15/1 -> Delay288/1
  relational16/1 -> Delay286/1
  [adc_lower_threshold] -> relational16/2
  [adc_upper_threshold] -> relational15/2
  Delay283/1 -> adc0_threshold_acc/1(out_reg)
  Register6/1 -> relational15/1, Delay284/1, relational16/1
  Delay284/1 -> adc1_threshold_acc/1(out_reg)
  Delay292/1 -> logical39/1
  Delay288/1 -> logical39/2
  Delay290/1 -> logical1/1
  Delay286/1 -> logical1/2
  logical39/1 -> Delay295/1
  logical1/1 -> Delay296/1
  Delay294/1 -> [adc_over_threshold], adc_over_threshold/1(out_reg)
  Delay293/1 -> [adc_under_threshold], adc_under_threshold/1(out_reg)
  Delay295/1 -> negedge_delay2/1(in)
  Delay296/1 -> negedge_delay1/1(in)
  negedge_delay1/1(out) -> Slice36/1
  negedge_delay2/1(out) -> Slice34/1
  reinterpret10/1 -> Delay269/1
  reinterpret11/1 -> Delay280/1
  Slice34/1 -> Delay294/1
  Slice36/1 -> Delay293/1
  Delay285/1 -> Register6/2
  Delay282/1 -> Register6/1
  Delay261/1 -> Register3/2
  Delay271/1 -> Register3/1
  Reinterpret12/1 -> Delay270/1
  Reinterpret13/1 -> Delay281/1
  [adc_threshold_acc_trig] -> Delay261/1, accumulator/2
  [adc_threshold_acc_trig] -> Delay285/1, accumulator1/2
  [adc_over_threshold] -> Delay297/1
  Delay297/1 -> Delay39/1
  [adc_under_threshold] -> Delay298/1
  Delay298/1 -> Delay44/1
  katadc/1(data0_0) -> Delay179/1
  katadc/2(data0_1) -> Delay180/1
  katadc/3(data0_2) -> Delay181/1
  katadc/4(data0_3) -> Delay182/1
  katadc/6(data1_0) -> Delay184/1
  katadc/7(data1_1) -> Delay185/1
  katadc/8(data1_2) -> Delay186/1
  katadc/9(data1_3) -> Delay187/1
  katadc/10(or1) -> Delay188/1
  katadc/5(or0) -> Delay183/1
  Delay179/1 -> Delay238/1
  Delay180/1 -> Delay254/1
  Delay181/1 -> Delay255/1
  Delay182/1 -> Delay256/1
  Delay183/1 -> [adc0_or]
  Delay184/1 -> Delay257/1
  Delay185/1 -> Delay258/1
  Delay186/1 -> Delay259/1
  Delay187/1 -> Delay260/1
  Delay188/1 -> [adc1_or]
  Delay238/1 -> [adc_data0_0]
  Delay254/1 -> [adc_data0_1]
  Delay255/1 -> [adc_data0_2]
  Delay256/1 -> [adc_data0_3]
  Delay257/1 -> [adc_data1_0]
  Delay258/1 -> [adc_data1_1]
  Delay259/1 -> [adc_data1_2]
  Delay260/1 -> [adc_data1_3]
  Delay54/1 -> pfb_fir_real/2(pol1_in1)
  Delay55/1 -> pfb_fir_real/3(pol1_in2)
  Delay198/1 -> pfb_fir_real/4(pol1_in3)
  Delay249/1 -> pfb_fir_real/5(pol1_in4)
  [adc_data0_0] -> Delay54/1
  [adc_data0_1] -> Delay55/1
  [adc_data0_2] -> Delay198/1
  [adc_data0_3] -> Delay249/1
  Delay253/1 -> pfb_fir_real1/5(pol1_in4)
  Delay252/1 -> pfb_fir_real1/4(pol1_in3)
  Delay251/1 -> pfb_fir_real1/3(pol1_in2)
  Delay250/1 -> pfb_fir_real1/2(pol1_in1)
  [adc_data1_0] -> Delay250/1
  [adc_data1_1] -> Delay251/1
  [adc_data1_2] -> Delay252/1
  [adc_data1_3] -> Delay253/1
